simulink model "ProcessNetworkSimulation"  (R2015b)
settings: Solver=VariableStepAuto  StartTime=0.0  StopTime=1000.0  RelTol=1e-3
libraries: simulink x1, simeventslib x1
(part 1 of 21)
settings Model: Creator=tsprock3  LastModifiedBy=tsprock3

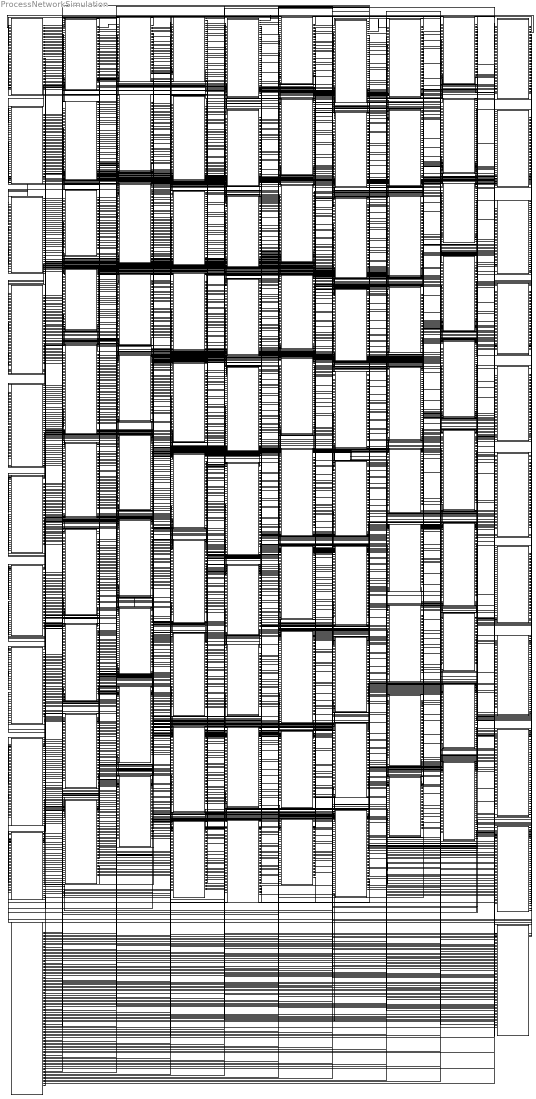
== system ProcessNetworkSimulation ==
  Arrival_Process : Subsystem
  Departure_Process : Subsystem
  Process_1 : Subsystem
  Process_10 : Subsystem
  Process_100 : Subsystem
  Process_11 : Subsystem
  Process_12 : Subsystem
  Process_13 : Subsystem
  Process_14 : Subsystem
  Process_15 : Subsystem
  Process_16 : Subsystem
  Process_17 : Subsystem
  Process_18 : Subsystem
  Process_19 : Subsystem
  Process_2 : Subsystem
  Process_20 : Subsystem
  Process_21 : Subsystem
  Process_22 : Subsystem
  Process_23 : Subsystem
  Process_24 : Subsystem
  Process_25 : Subsystem
  Process_26 : Subsystem
  Process_27 : Subsystem
  Process_28 : Subsystem
  Process_29 : Subsystem
  Process_3 : Subsystem
  Process_30 : Subsystem
  Process_31 : Subsystem
  Process_32 : Subsystem
  Process_33 : Subsystem
  Process_34 : Subsystem
  Process_35 : Subsystem
  Process_36 : Subsystem
  Process_37 : Subsystem
  Process_38 : Subsystem
  Process_39 : Subsystem
  Process_4 : Subsystem
  Process_40 : Subsystem
  Process_41 : Subsystem
  Process_42 : Subsystem
  Process_43 : Subsystem
  Process_44 : Subsystem
  Process_45 : Subsystem
  Process_46 : Subsystem
  Process_47 : Subsystem
  Process_48 : Subsystem
  Process_49 : Subsystem
  Process_5 : Subsystem
  Process_50 : Subsystem
  Process_51 : Subsystem
  Process_52 : Subsystem
  Process_53 : Subsystem
  Process_54 : Subsystem
  Process_55 : Subsystem
  Process_56 : Subsystem
  Process_57 : Subsystem
  Process_58 : Subsystem
  Process_59 : Subsystem
  Process_6 : Subsystem
  Process_60 : Subsystem
  Process_61 : Subsystem
  Process_62 : Subsystem
  Process_63 : Subsystem
  Process_64 : Subsystem
  Process_65 : Subsystem
  Process_66 : Subsystem
  Process_67 : Subsystem
  Process_68 : Subsystem
  Process_69 : Subsystem
  Process_7 : Subsystem
  Process_70 : Subsystem
  Process_71 : Subsystem
  Process_72 : Subsystem
  Process_73 : Subsystem
  Process_74 : Subsystem
  Process_75 : Subsystem
  Process_76 : Subsystem
  Process_77 : Subsystem
  Process_78 : Subsystem
  Process_79 : Subsystem
  Process_8 : Subsystem
  Process_80 : Subsystem
  Process_81 : Subsystem
  Process_82 : Subsystem
  Process_83 : Subsystem
  Process_84 : Subsystem
  Process_85 : Subsystem
  Process_86 : Subsystem
  Process_87 : Subsystem
  Process_88 : Subsystem
  Process_89 : Subsystem
  Process_9 : Subsystem
  Process_90 : Subsystem
  Process_91 : Subsystem
  Process_92 : Subsystem
  Process_93 : Subsystem
  Process_94 : Subsystem
  Process_95 : Subsystem
  Process_96 : Subsystem
  Process_97 : Subsystem
  Process_98 : Subsystem
  Process_99 : Subsystem
  connections:
  Process_1/RConn1 -- Process_1/LConn1
  Process_1/RConn2 -- Process_2/LConn1
  Process_1/RConn3 -- Process_4/LConn1
  Process_1/RConn4 -- Process_8/LConn1
  Process_1/RConn5 -- Process_10/LConn1
  Process_1/RConn6 -- Process_11/LConn1
  Process_1/RConn7 -- Process_16/LConn1
  Process_1/RConn8 -- Process_18/LConn1
  Process_1/RConn9 -- Process_23/LConn1
  Process_1/RConn10 -- Process_24/LConn1
  Process_1/RConn11 -- Process_25/LConn1
  Process_1/RConn12 -- Process_30/LConn1
  Process_1/RConn13 -- Process_33/LConn1
  Process_1/RConn14 -- Process_35/LConn1
  Process_1/RConn15 -- Process_38/LConn1
  Process_1/RConn16 -- Process_40/LConn1
  Process_1/RConn17 -- Process_45/LConn1
  Process_1/RConn18 -- Process_48/LConn1
  Process_1/RConn19 -- Process_54/LConn1
  Process_1/RConn20 -- Process_57/LConn1
  Process_1/RConn21 -- Process_58/LConn1
  Process_1/RConn22 -- Process_59/LConn1
  Process_1/RConn23 -- Process_64/LConn1
  Process_1/RConn24 -- Process_65/LConn1
  Process_1/RConn25 -- Process_67/LConn1
  Process_1/RConn26 -- Process_69/LConn1
  Process_1/RConn27 -- Process_71/LConn1
  Process_1/RConn28 -- Process_72/LConn1
  Process_1/RConn29 -- Process_74/LConn1
  Process_1/RConn30 -- Process_77/LConn1
  Process_1/RConn31 -- Process_81/LConn1
  Process_1/RConn32 -- Process_83/LConn1
  Process_1/RConn33 -- Process_93/LConn1
  Process_1/RConn34 -- Process_97/LConn1
  Process_1/RConn35 -- Process_99/LConn1
  Process_1/RConn36 -- Process_100/LConn1
  Process_2/RConn1 -- Process_1/LConn2
  Process_2/RConn2 -- Process_6/LConn1
  Process_2/RConn3 -- Process_15/LConn1
  Process_2/RConn4 -- Process_18/LConn2
  Process_2/RConn5 -- Process_19/LConn1
  Process_2/RConn6 -- Process_20/LConn1
  Process_2/RConn7 -- Process_22/LConn1
  Process_2/RConn8 -- Process_27/LConn1
  Process_2/RConn9 -- Process_30/LConn2
  Process_2/RConn10 -- Process_32/LConn1
  Process_2/RConn11 -- Process_33/LConn2
  Process_2/RConn12 -- Process_42/LConn1
  Process_2/RConn13 -- Process_45/LConn2
  Process_2/RConn14 -- Process_46/LConn1
  Process_2/RConn15 -- Process_52/LConn1
  Process_2/RConn16 -- Process_54/LConn2
  Process_2/RConn17 -- Process_56/LConn1
  Process_2/RConn18 -- Process_58/LConn2
  Process_2/RConn19 -- Process_59/LConn2
  Process_2/RConn20 -- Process_60/LConn1
  Process_2/RConn21 -- Process_67/LConn2
  Process_2/RConn22 -- Process_69/LConn2
  Process_2/RConn23 -- Process_82/LConn1
  Process_2/RConn24 -- Process_85/LConn1
  Process_2/RConn25 -- Process_91/LConn1
  Process_2/RConn26 -- Process_92/LConn1
  Process_2/RConn27 -- Process_93/LConn2
  Process_2/RConn28 -- Process_95/LConn1
  Process_2/RConn29 -- Process_96/LConn1
  Process_2/RConn30 -- Process_98/LConn1
  Process_2/RConn31 -- Process_99/LConn2
  Process_3/RConn1 -- Process_6/LConn2
  Process_3/RConn2 -- Process_11/LConn2
  Process_3/RConn3 -- Process_16/LConn2
  Process_3/RConn4 -- Process_28/LConn1
  Process_3/RConn5 -- Process_34/LConn1
  Process_3/RConn6 -- Process_35/LConn2
  Process_3/RConn7 -- Process_43/LConn1
  Process_3/RConn8 -- Process_44/LConn1
  Process_3/RConn9 -- Process_45/LConn3
  Process_3/RConn10 -- Process_51/LConn1
  Process_3/RConn11 -- Process_52/LConn2
  Process_3/RConn12 -- Process_55/LConn1
  Process_3/RConn13 -- Process_60/LConn2
  Process_3/RConn14 -- Process_62/LConn1
  Process_3/RConn15 -- Process_66/LConn1
  Process_3/RConn16 -- Process_68/LConn1
  Process_3/RConn17 -- Process_71/LConn2
  Process_3/RConn18 -- Process_75/LConn1
  Process_3/RConn19 -- Process_77/LConn2
  Process_3/RConn20 -- Process_79/LConn1
  Process_3/RConn21 -- Process_80/LConn1
  Process_3/RConn22 -- Process_83/LConn2
  Process_3/RConn23 -- Process_85/LConn2
  Process_3/RConn24 -- Process_88/LConn1
  Process_3/RConn25 -- Process_92/LConn2
  Process_3/RConn26 -- Process_95/LConn2
  Process_3/RConn27 -- Process_97/LConn2
  Process_3/RConn28 -- Process_98/LConn2
  Process_3/RConn29 -- Process_99/LConn3
  Process_3/RConn30 -- Process_100/LConn2
  Process_4/RConn1 -- Process_5/LConn1
  Process_4/RConn2 -- Process_6/LConn3
  Process_4/RConn3 -- Process_9/LConn1
  Process_4/RConn4 -- Process_11/LConn3
  Process_4/RConn5 -- Process_20/LConn2
  Process_4/RConn6 -- Process_22/LConn2
  Process_4/RConn7 -- Process_23/LConn2
  Process_4/RConn8 -- Process_29/LConn1
  Process_4/RConn9 -- Process_30/LConn3
  Process_4/RConn10 -- Process_33/LConn3
  Process_4/RConn11 -- Process_37/LConn1
  Process_4/RConn12 -- Process_39/LConn1
  Process_4/RConn13 -- Process_41/LConn1
  Process_4/RConn14 -- Process_42/LConn2
  Process_4/RConn15 -- Process_43/LConn2
  Process_4/RConn16 -- Process_44/LConn2
  Process_4/RConn17 -- Process_47/LConn1
  Process_4/RConn18 -- Process_49/LConn1
  Process_4/RConn19 -- Process_50/LConn1
  Process_4/RConn20 -- Process_53/LConn1
  Process_4/RConn21 -- Process_57/LConn2
  Process_4/RConn22 -- Process_64/LConn2
  Process_4/RConn23 -- Process_70/LConn1
  Process_4/RConn24 -- Process_72/LConn2
  Process_4/RConn25 -- Process_74/LConn2
  Process_4/RConn26 -- Process_77/LConn3
  Process_4/RConn27 -- Process_81/LConn2
  Process_4/RConn28 -- Process_83/LConn3
  Process_4/RConn29 -- Process_84/LConn1
  Process_4/RConn30 -- Process_86/LConn1
  Process_4/RConn31 -- Process_89/LConn1
  Process_4/RConn32 -- Process_90/LConn1
  Process_4/RConn33 -- Process_91/LConn2
  Process_4/RConn34 -- Process_94/LConn1
  Process_4/RConn35 -- Process_95/LConn3
  Process_4/RConn36 -- Process_100/LConn3
  Process_5/RConn1 -- Process_5/LConn2
  Process_5/RConn2 -- Process_8/LConn2
  Process_5/RConn3 -- Process_9/LConn2
  Process_5/RConn4 -- Process_13/LConn1
  Process_5/RConn5 -- Process_15/LConn2
  Process_5/RConn6 -- Process_16/LConn3
  Process_5/RConn7 -- Process_17/LConn1
  Process_5/RConn8 -- Process_21/LConn1
  Process_5/RConn9 -- Process_30/LConn4
  Process_5/RConn10 -- Process_32/LConn2
  Process_5/RConn11 -- Process_35/LConn3
  Process_5/RConn12 -- Process_37/LConn2
  Process_5/RConn13 -- Process_38/LConn2
  Process_5/RConn14 -- Process_45/LConn4
  Process_5/RConn15 -- Process_48/LConn2
  Process_5/RConn16 -- Process_53/LConn2
  Process_5/RConn17 -- Process_56/LConn2
  Process_5/RConn18 -- Process_58/LConn3
  Process_5/RConn19 -- Process_59/LConn3
  Process_5/RConn20 -- Process_62/LConn2
  Process_5/RConn21 -- Process_63/LConn1
  Process_5/RConn22 -- Process_64/LConn3
  Process_5/RConn23 -- Process_68/LConn2
  Process_5/RConn24 -- Process_72/LConn3
  Process_5/RConn25 -- Process_75/LConn2
  Process_5/RConn26 -- Process_76/LConn1
  Process_5/RConn27 -- Process_79/LConn2
  Process_5/RConn28 -- Process_81/LConn3
  Process_5/RConn29 -- Process_82/LConn2
  Process_5/RConn30 -- Process_83/LConn4
  Process_5/RConn31 -- Process_88/LConn2
  Process_5/RConn32 -- Process_90/LConn2
  Process_5/RConn33 -- Process_94/LConn2
  Process_5/RConn34 -- Process_95/LConn4
  Process_5/RConn35 -- Process_96/LConn2
  Process_6/RConn1 -- Process_1/LConn3
  Process_6/RConn2 -- Process_2/LConn2
  Process_6/RConn3 -- Process_4/LConn2
  Process_6/RConn4 -- Process_5/LConn3
  Process_6/RConn5 -- Process_6/LConn4
  Process_6/RConn6 -- Process_7/LConn1
  Process_6/RConn7 -- Process_8/LConn3
  Process_6/RConn8 -- Process_11/LConn4
  Process_6/RConn9 -- Process_14/LConn1
  Process_6/RConn10 -- Process_16/LConn4
  Process_6/RConn11 -- Process_17/LConn2
  Process_6/RConn12 -- Process_18/LConn3
  Process_6/RConn13 -- Process_19/LConn2
  Process_6/RConn14 -- Process_21/LConn2
  Process_6/RConn15 -- Process_29/LConn2
  Process_6/RConn16 -- Process_36/LConn1
  Process_6/RConn17 -- Process_38/LConn3
  Process_6/RConn18 -- Process_43/LConn3
  Process_6/RConn19 -- Process_44/LConn3
  Process_6/RConn20 -- Process_46/LConn2
  Process_6/RConn21 -- Process_47/LConn2
  Process_6/RConn22 -- Process_50/LConn2
  Process_6/RConn23 -- Process_58/LConn4
  Process_6/RConn24 -- Process_59/LConn4
  Process_6/RConn25 -- Process_60/LConn3
  Process_6/RConn26 -- Process_61/LConn1
  Process_6/RConn27 -- Process_63/LConn2
  Process_6/RConn28 -- Process_66/LConn2
  Process_6/RConn29 -- Process_67/LConn3
  Process_6/RConn30 -- Process_68/LConn3
  Process_6/RConn31 -- Process_77/LConn4
  Process_6/RConn32 -- Process_83/LConn5
  Process_6/RConn33 -- Process_85/LConn3
  Process_6/RConn34 -- Process_86/LConn2
  Process_6/RConn35 -- Process_89/LConn2
  Process_6/RConn36 -- Process_90/LConn3
  Process_6/RConn37 -- Process_97/LConn3
  Process_6/RConn38 -- Process_98/LConn3
  Process_7/RConn1 -- Process_2/LConn3
  Process_7/RConn2 -- Process_3/LConn1
  Process_7/RConn3 -- Process_7/LConn2
  Process_7/RConn4 -- Process_9/LConn3
  Process_7/RConn5 -- Process_16/LConn5
  Process_7/RConn6 -- Process_18/LConn4
  Process_7/RConn7 -- Process_20/LConn3
  Process_7/RConn8 -- Process_21/LConn3
  Process_7/RConn9 -- Process_27/LConn2
  Process_7/RConn10 -- Process_29/LConn3
  Process_7/RConn11 -- Process_32/LConn3
  Process_7/RConn12 -- Process_33/LConn4
  Process_7/RConn13 -- Process_35/LConn4
  Process_7/RConn14 -- Process_38/LConn4
  Process_7/RConn15 -- Process_39/LConn2
  Process_7/RConn16 -- Process_40/LConn2
  Process_7/RConn17 -- Process_41/LConn2
  Process_7/RConn18 -- Process_42/LConn3
  Process_7/RConn19 -- Process_46/LConn3
  Process_7/RConn20 -- Process_47/LConn3
  Process_7/RConn21 -- Process_50/LConn3
  Process_7/RConn22 -- Process_51/LConn2
  Process_7/RConn23 -- Process_52/LConn3
  Process_7/RConn24 -- Process_56/LConn3
  Process_7/RConn25 -- Process_59/LConn5
  Process_7/RConn26 -- Process_60/LConn4
  Process_7/RConn27 -- Process_61/LConn2
  Process_7/RConn28 -- Process_62/LConn3
  Process_7/RConn29 -- Process_64/LConn4
  Process_7/RConn30 -- Process_66/LConn3
  Process_7/RConn31 -- Process_67/LConn4
  Process_7/RConn32 -- Process_74/LConn3
  Process_7/RConn33 -- Process_75/LConn3
  Process_7/RConn34 -- Process_77/LConn5
  Process_7/RConn35 -- Process_79/LConn3
  Process_7/RConn36 -- Process_80/LConn2
  Process_7/RConn37 -- Process_82/LConn3
  Process_7/RConn38 -- Process_83/LConn6
  Process_7/RConn39 -- Process_89/LConn3
  Process_7/RConn40 -- Process_90/LConn4
  Process_7/RConn41 -- Process_93/LConn3
  Process_8/RConn1 -- Process_3/LConn2
  Process_8/RConn2 -- Process_6/LConn5
  Process_8/RConn3 -- Process_12/LConn1
  Process_8/RConn4 -- Process_13/LConn2
  Process_8/RConn5 -- Process_16/LConn6
  Process_8/RConn6 -- Process_23/LConn3
  Process_8/RConn7 -- Process_27/LConn3
  Process_8/RConn8 -- Process_30/LConn5
  Process_8/RConn9 -- Process_36/LConn2
  Process_8/RConn10 -- Process_37/LConn3
  Process_8/RConn11 -- Process_38/LConn5
  Process_8/RConn12 -- Process_41/LConn3
  Process_8/RConn13 -- Process_42/LConn4
  Process_8/RConn14 -- Process_43/LConn4
  Process_8/RConn15 -- Process_46/LConn4
  Process_8/RConn16 -- Process_50/LConn4
  Process_8/RConn17 -- Process_53/LConn3
  Process_8/RConn18 -- Process_54/LConn3
  Process_8/RConn19 -- Process_56/LConn4
  Process_8/RConn20 -- Process_60/LConn5
  Process_8/RConn21 -- Process_68/LConn4
  Process_8/RConn22 -- Process_71/LConn3
  Process_8/RConn23 -- Process_73/LConn1
  Process_8/RConn24 -- Process_74/LConn4
  Process_8/RConn25 -- Process_76/LConn2
  Process_8/RConn26 -- Process_77/LConn6
  Process_8/RConn27 -- Process_79/LConn4
  Process_8/RConn28 -- Process_80/LConn3
  Process_8/RConn29 -- Process_86/LConn3
  Process_8/RConn30 -- Process_90/LConn5
  Process_8/RConn31 -- Process_91/LConn3
  Process_8/RConn32 -- Process_95/LConn5
  Process_8/RConn33 -- Process_97/LConn4
  Process_9/RConn1 -- Process_2/LConn4
  Process_9/RConn2 -- Process_3/LConn3
  Process_9/RConn3 -- Process_4/LConn3
  Process_9/RConn4 -- Process_6/LConn6
  Process_9/RConn5 -- Process_10/LConn2
  Process_9/RConn6 -- Process_11/LConn5
  Process_9/RConn7 -- Process_13/LConn3
  Process_9/RConn8 -- Process_14/LConn2
  Process_9/RConn9 -- Process_15/LConn3
  Process_9/RConn10 -- Process_23/LConn4
  Process_9/RConn11 -- Process_24/LConn2
  Process_9/RConn12 -- Process_26/LConn1
  Process_9/RConn13 -- Process_27/LConn4
  Process_9/RConn14 -- Process_28/LConn2
  Process_9/RConn15 -- Process_30/LConn6
  Process_9/RConn16 -- Process_31/LConn1
  Process_9/RConn17 -- Process_32/LConn4
  Process_9/RConn18 -- Process_34/LConn2
  Process_9/RConn19 -- Process_36/LConn3
  Process_9/RConn20 -- Process_37/LConn4
  Process_9/RConn21 -- Process_38/LConn6
  Process_9/RConn22 -- Process_40/LConn3
  Process_9/RConn23 -- Process_41/LConn4
  Process_9/RConn24 -- Process_42/LConn5
  Process_9/RConn25 -- Process_44/LConn4
  Process_9/RConn26 -- Process_49/LConn2
  Process_9/RConn27 -- Process_55/LConn2
  Process_9/RConn28 -- Process_56/LConn5
  Process_9/RConn29 -- Process_58/LConn5
  Process_9/RConn30 -- Process_61/LConn3
  Process_9/RConn31 -- Process_62/LConn4
  Process_9/RConn32 -- Process_65/LConn2
  Process_9/RConn33 -- Process_71/LConn4
  Process_9/RConn34 -- Process_76/LConn3
  Process_9/RConn35 -- Process_80/LConn4
  Process_9/RConn36 -- Process_82/LConn4
  Process_9/RConn37 -- Process_83/LConn7
  Process_9/RConn38 -- Process_88/LConn3
  Process_9/RConn39 -- Process_92/LConn3
  Process_9/RConn40 -- Process_93/LConn4
  Process_9/RConn41 -- Process_98/LConn4
  Process_9/RConn42 -- Process_99/LConn4
  Process_10/RConn1 -- Process_2/LConn5
  Process_10/RConn2 -- Process_4/LConn4
  Process_10/RConn3 -- Process_5/LConn4
  Process_10/RConn4 -- Process_8/LConn4
  Process_10/RConn5 -- Process_9/LConn4
  Process_10/RConn6 -- Process_11/LConn6
  Process_10/RConn7 -- Process_14/LConn3
  Process_10/RConn8 -- Process_18/LConn5
  Process_10/RConn9 -- Process_22/LConn3
  Process_10/RConn10 -- Process_24/LConn3
  Process_10/RConn11 -- Process_25/LConn2
  Process_10/RConn12 -- Process_26/LConn2
  Process_10/RConn13 -- Process_29/LConn4
  Process_10/RConn14 -- Process_33/LConn5
  Process_10/RConn15 -- Process_37/LConn5
  Process_10/RConn16 -- Process_38/LConn7
  Process_10/RConn17 -- Process_41/LConn5
  Process_10/RConn18 -- Process_42/LConn6
  Process_10/RConn19 -- Process_43/LConn5
  Process_10/RConn20 -- Process_48/LConn3
  Process_10/RConn21 -- Process_49/LConn3
  Process_10/RConn22 -- Process_50/LConn5
  Process_10/RConn23 -- Process_59/LConn6
  Process_10/RConn24 -- Process_63/LConn3
  Process_10/RConn25 -- Process_68/LConn5
  Process_10/RConn26 -- Process_70/LConn2
  Process_10/RConn27 -- Process_72/LConn4
  Process_10/RConn28 -- Process_75/LConn4
  Process_10/RConn29 -- Process_76/LConn4
  Process_10/RConn30 -- Process_79/LConn5
  Process_10/RConn31 -- Process_80/LConn5
  Process_10/RConn32 -- Process_81/LConn4
  Process_10/RConn33 -- Process_83/LConn8
  Process_10/RConn34 -- Process_84/LConn2
  Process_10/RConn35 -- Process_89/LConn4
  Process_10/RConn36 -- Process_90/LConn6
  Process_10/RConn37 -- Process_91/LConn4
  Process_10/RConn38 -- Process_92/LConn4
  Process_10/RConn39 -- Process_93/LConn5
  Process_10/RConn40 -- Process_95/LConn6
  Process_11/RConn1 -- Process_6/LConn7
  Process_11/RConn2 -- Process_7/LConn3
  Process_11/RConn3 -- Process_9/LConn5
  Process_11/RConn4 -- Process_13/LConn4
  Process_11/RConn5 -- Process_15/LConn4
  Process_11/RConn6 -- Process_18/LConn6
  Process_11/RConn7 -- Process_21/LConn4
  Process_11/RConn8 -- Process_28/LConn3
  Process_11/RConn9 -- Process_29/LConn5
  Process_11/RConn10 -- Process_33/LConn6
  Process_11/RConn11 -- Process_36/LConn4
  Process_11/RConn12 -- Process_40/LConn4
  Process_11/RConn13 -- Process_41/LConn6
  Process_11/RConn14 -- Process_42/LConn7
  Process_11/RConn15 -- Process_44/LConn5
  Process_11/RConn16 -- Process_45/LConn5
  Process_11/RConn17 -- Process_46/LConn5
  Process_11/RConn18 -- Process_47/LConn4
  Process_11/RConn19 -- Process_49/LConn4
  Process_11/RConn20 -- Process_53/LConn4
  Process_11/RConn21 -- Process_55/LConn3
  Process_11/RConn22 -- Process_59/LConn7
  Process_11/RConn23 -- Process_61/LConn4
  Process_11/RConn24 -- Process_67/LConn5
  Process_11/RConn25 -- Process_68/LConn6
  Process_11/RConn26 -- Process_70/LConn3
  Process_11/RConn27 -- Process_72/LConn5
  Process_11/RConn28 -- Process_73/LConn2
  Process_11/RConn29 -- Process_74/LConn5
  Process_11/RConn30 -- Process_77/LConn7
  Process_11/RConn31 -- Process_82/LConn5
  Process_11/RConn32 -- Process_83/LConn9
  Process_11/RConn33 -- Process_93/LConn6
  Process_11/RConn34 -- Process_96/LConn3
  Process_11/RConn35 -- Process_99/LConn5
  Process_11/RConn36 -- Process_100/LConn4
  Process_12/RConn1 -- Process_1/LConn4
  Process_12/RConn2 -- Process_4/LConn5
  Process_12/RConn3 -- Process_6/LConn8
  Process_12/RConn4 -- Process_7/LConn4
  Process_12/RConn5 -- Process_9/LConn6
  Process_12/RConn6 -- Process_10/LConn3
  Process_12/RConn7 -- Process_13/LConn5
  Process_12/RConn8 -- Process_14/LConn4
  Process_12/RConn9 -- Process_16/LConn7
  Process_12/RConn10 -- Process_19/LConn3
  Process_12/RConn11 -- Process_23/LConn5
  Process_12/RConn12 -- Process_28/LConn4
  Process_12/RConn13 -- Process_30/LConn7
  Process_12/RConn14 -- Process_35/LConn5
  Process_12/RConn15 -- Process_36/LConn5
  Process_12/RConn16 -- Process_41/LConn7
  Process_12/RConn17 -- Process_44/LConn6
  Process_12/RConn18 -- Process_46/LConn6
  Process_12/RConn19 -- Process_47/LConn5
  Process_12/RConn20 -- Process_50/LConn6
  Process_12/RConn21 -- Process_52/LConn4
  Process_12/RConn22 -- Process_55/LConn4
  Process_12/RConn23 -- Process_56/LConn6
  Process_12/RConn24 -- Process_57/LConn3
  Process_12/RConn25 -- Process_58/LConn6
  Process_12/RConn26 -- Process_61/LConn5
  Process_12/RConn27 -- Process_62/LConn5
  Process_12/RConn28 -- Process_65/LConn3
  Process_12/RConn29 -- Process_71/LConn5
  Process_12/RConn30 -- Process_72/LConn6
  Process_12/RConn31 -- Process_73/LConn3
  Process_12/RConn32 -- Process_74/LConn6
  Process_12/RConn33 -- Process_78/LConn1
  Process_12/RConn34 -- Process_80/LConn6
  Process_12/RConn35 -- Process_83/LConn10
  Process_12/RConn36 -- Process_89/LConn5
  Process_12/RConn37 -- Process_91/LConn5
  Process_12/RConn38 -- Process_92/LConn5
  Process_12/RConn39 -- Process_93/LConn7
  Process_12/RConn40 -- Process_99/LConn6
  Process_13/RConn1 -- Process_6/LConn9
  Process_13/RConn2 -- Process_7/LConn5
  Process_13/RConn3 -- Process_11/LConn7
  Process_13/RConn4 -- Process_17/LConn3
  Process_13/RConn5 -- Process_18/LConn7
  Process_13/RConn6 -- Process_19/LConn4
  Process_13/RConn7 -- Process_20/LConn4
  Process_13/RConn8 -- Process_22/LConn4
  Process_13/RConn9 -- Process_24/LConn4
  Process_13/RConn10 -- Process_25/LConn3
  Process_13/RConn11 -- Process_26/LConn3
  Process_13/RConn12 -- Process_28/LConn5
  Process_13/RConn13 -- Process_30/LConn8
  Process_13/RConn14 -- Process_31/LConn2
  Process_13/RConn15 -- Process_33/LConn7
  Process_13/RConn16 -- Process_35/LConn6
  Process_13/RConn17 -- Process_36/LConn6
  Process_13/RConn18 -- Process_38/LConn8
  Process_13/RConn19 -- Process_39/LConn3
  Process_13/RConn20 -- Process_40/LConn5
  Process_13/RConn21 -- Process_45/LConn6
  Process_13/RConn22 -- Process_48/LConn4
  Process_13/RConn23 -- Process_50/LConn7
  Process_13/RConn24 -- Process_55/LConn5
  Process_13/RConn25 -- Process_62/LConn6
  Process_13/RConn26 -- Process_65/LConn4
  Process_13/RConn27 -- Process_66/LConn4
  Process_13/RConn28 -- Process_68/LConn7
  Process_13/RConn29 -- Process_69/LConn3
  Process_13/RConn30 -- Process_70/LConn4
  Process_13/RConn31 -- Process_71/LConn6
  Process_13/RConn32 -- Process_72/LConn7
  Process_13/RConn33 -- Process_75/LConn5
  Process_13/RConn34 -- Process_76/LConn5
  Process_13/RConn35 -- Process_80/LConn7
  Process_13/RConn36 -- Process_82/LConn6
  Process_13/RConn37 -- Process_88/LConn4
  Process_13/RConn38 -- Process_89/LConn6
  Process_13/RConn39 -- Process_97/LConn5
  Process_13/RConn40 -- Process_98/LConn5
  Process_13/RConn41 -- Process_99/LConn7
  Process_14/RConn1 -- Process_3/LConn4
  Process_14/RConn2 -- Process_6/LConn10
  Process_14/RConn3 -- Process_7/LConn6
  Process_14/RConn4 -- Process_8/LConn5
  Process_14/RConn5 -- Process_9/LConn7
  Process_14/RConn6 -- Process_12/LConn2
  Process_14/RConn7 -- Process_13/LConn6
  Process_14/RConn8 -- Process_16/LConn8
  Process_14/RConn9 -- Process_18/LConn8
  Process_14/RConn10 -- Process_21/LConn5
  Process_14/RConn11 -- Process_23/LConn6
  Process_14/RConn12 -- Process_25/LConn4
  Process_14/RConn13 -- Process_26/LConn4
  Process_14/RConn14 -- Process_27/LConn5
  Process_14/RConn15 -- Process_29/LConn6
  Process_14/RConn16 -- Process_31/LConn3
  Process_14/RConn17 -- Process_40/LConn6
  Process_14/RConn18 -- Process_41/LConn8
  Process_14/RConn19 -- Process_43/LConn6
  Process_14/RConn20 -- Process_50/LConn8
  Process_14/RConn21 -- Process_51/LConn3
  Process_14/RConn22 -- Process_53/LConn5
  Process_14/RConn23 -- Process_56/LConn7
  Process_14/RConn24 -- Process_57/LConn4
  Process_14/RConn25 -- Process_58/LConn7
  Process_14/RConn26 -- Process_60/LConn6
  Process_14/RConn27 -- Process_61/LConn6
  Process_14/RConn28 -- Process_65/LConn5
  Process_14/RConn29 -- Process_66/LConn5
  Process_14/RConn30 -- Process_71/LConn7
  Process_14/RConn31 -- Process_74/LConn7
  Process_14/RConn32 -- Process_82/LConn7
  Process_14/RConn33 -- Process_83/LConn11
  Process_14/RConn34 -- Process_84/LConn3
  Process_14/RConn35 -- Process_89/LConn7
  Process_14/RConn36 -- Process_90/LConn7
  Process_14/RConn37 -- Process_91/LConn6
  Process_14/RConn38 -- Process_98/LConn6
  Process_14/RConn39 -- Process_99/LConn8
  Process_15/RConn1 -- Process_3/LConn5
  Process_15/RConn2 -- Process_4/LConn6
  Process_15/RConn3 -- Process_5/LConn5
  Process_15/RConn4 -- Process_15/LConn5
  Process_15/RConn5 -- Process_16/LConn9
  Process_15/RConn6 -- Process_17/LConn4
  Process_15/RConn7 -- Process_19/LConn5
  Process_15/RConn8 -- Process_25/LConn5
  Process_15/RConn9 -- Process_27/LConn6
  Process_15/RConn10 -- Process_30/LConn9
  Process_15/RConn11 -- Process_37/LConn6
  Process_15/RConn12 -- Process_39/LConn4
  Process_15/RConn13 -- Process_40/LConn7
  Process_15/RConn14 -- Process_41/LConn9
  Process_15/RConn15 -- Process_43/LConn7
  Process_15/RConn16 -- Process_46/LConn7
  Process_15/RConn17 -- Process_48/LConn5
  Process_15/RConn18 -- Process_49/LConn5
  Process_15/RConn19 -- Process_50/LConn9
  Process_15/RConn20 -- Process_54/LConn4
  Process_15/RConn21 -- Process_55/LConn6
  Process_15/RConn22 -- Process_56/LConn8
  Process_15/RConn23 -- Process_59/LConn8
  Process_15/RConn24 -- Process_60/LConn7
  Process_15/RConn25 -- Process_61/LConn7
  Process_15/RConn26 -- Process_63/LConn4
  Process_15/RConn27 -- Process_65/LConn6
  Process_15/RConn28 -- Process_66/LConn6
  Process_15/RConn29 -- Process_69/LConn4
  Process_15/RConn30 -- Process_73/LConn4
  Process_15/RConn31 -- Process_75/LConn6
  Process_15/RConn32 -- Process_82/LConn8
  Process_15/RConn33 -- Process_86/LConn4
  Process_15/RConn34 -- Process_87/LConn1
  Process_15/RConn35 -- Process_94/LConn3
  Process_15/RConn36 -- Process_98/LConn7
  Process_15/RConn37 -- Process_99/LConn9
  Process_16/RConn1 -- Process_4/LConn7
  Process_16/RConn2 -- Process_8/LConn6
  Process_16/RConn3 -- Process_9/LConn8
  Process_16/RConn4 -- Process_10/LConn4
  Process_16/RConn5 -- Process_12/LConn3
  Process_16/RConn6 -- Process_13/LConn7
  Process_16/RConn7 -- Process_16/LConn10
  Process_16/RConn8 -- Process_17/LConn5
  Process_16/RConn9 -- Process_19/LConn6
  Process_16/RConn10 -- Process_22/LConn5
  Process_16/RConn11 -- Process_23/LConn7
  Process_16/RConn12 -- Process_25/LConn6
  Process_16/RConn13 -- Process_26/LConn5
  Process_16/RConn14 -- Process_30/LConn10
  Process_16/RConn15 -- Process_42/LConn8
  Process_16/RConn16 -- Process_48/LConn6
  Process_16/RConn17 -- Process_49/LConn6
  Process_16/RConn18 -- Process_50/LConn10
  Process_16/RConn19 -- Process_51/LConn4
  Process_16/RConn20 -- Process_52/LConn5
  Process_16/RConn21 -- Process_55/LConn7
  Process_16/RConn22 -- Process_57/LConn5
  Process_16/RConn23 -- Process_58/LConn8
  Process_16/RConn24 -- Process_60/LConn8
  Process_16/RConn25 -- Process_61/LConn8
  Process_16/RConn26 -- Process_66/LConn7
  Process_16/RConn27 -- Process_69/LConn5
  Process_16/RConn28 -- Process_71/LConn8
  Process_16/RConn29 -- Process_75/LConn7
  Process_16/RConn30 -- Process_79/LConn6
  Process_16/RConn31 -- Process_81/LConn5
  Process_16/RConn32 -- Process_82/LConn9
  Process_16/RConn33 -- Process_83/LConn12
  Process_16/RConn34 -- Process_86/LConn5
  Process_16/RConn35 -- Process_87/LConn2
  Process_16/RConn36 -- Process_94/LConn4
  Process_16/RConn37 -- Process_96/LConn4
  Process_16/RConn38 -- Process_98/LConn8
  Process_16/RConn39 -- Process_99/LConn10
  Process_17/RConn1 -- Process_1/LConn5
  Process_17/RConn2 -- Process_3/LConn6
  Process_17/RConn3 -- Process_7/LConn7
  Process_17/RConn4 -- Process_10/LConn5
  Process_17/RConn5 -- Process_14/LConn5
  Process_17/RConn6 -- Process_17/LConn6
  Process_17/RConn7 -- Process_22/LConn6
  Process_17/RConn8 -- Process_23/LConn8
  Process_17/RConn9 -- Process_26/LConn6
  Process_17/RConn10 -- Process_30/LConn11
  Process_17/RConn11 -- Process_33/LConn8
  Process_17/RConn12 -- Process_34/LConn3
  Process_17/RConn13 -- Process_38/LConn9
  Process_17/RConn14 -- Process_41/LConn10
  Process_17/RConn15 -- Process_53/LConn6
  Process_17/RConn16 -- Process_57/LConn6
  Process_17/RConn17 -- Process_58/LConn9
  Process_17/RConn18 -- Process_64/LConn5
  Process_17/RConn19 -- Process_70/LConn5
  Process_17/RConn20 -- Process_76/LConn6
  Process_17/RConn21 -- Process_79/LConn7
  Process_17/RConn22 -- Process_80/LConn8
  Process_17/RConn23 -- Process_82/LConn10
  Process_17/RConn24 -- Process_83/LConn13
  Process_17/RConn25 -- Process_89/LConn8
  Process_17/RConn26 -- Process_93/LConn8
  Process_17/RConn27 -- Process_94/LConn5
  Process_17/RConn28 -- Process_96/LConn5
  Process_17/RConn29 -- Process_97/LConn6
  Process_17/RConn30 -- Process_98/LConn9
  Process_17/RConn31 -- Process_99/LConn11
  Process_17/RConn32 -- Process_100/LConn5
  Process_18/RConn1 -- Process_2/LConn6
  Process_18/RConn2 -- Process_10/LConn6
  Process_18/RConn3 -- Process_15/LConn6
  Process_18/RConn4 -- Process_17/LConn7
  Process_18/RConn5 -- Process_21/LConn6
  Process_18/RConn6 -- Process_22/LConn7
  Process_18/RConn7 -- Process_26/LConn7
  Process_18/RConn8 -- Process_27/LConn7
  Process_18/RConn9 -- Process_28/LConn6
  Process_18/RConn10 -- Process_31/LConn4
  Process_18/RConn11 -- Process_32/LConn5
  Process_18/RConn12 -- Process_34/LConn4
  Process_18/RConn13 -- Process_36/LConn7
  Process_18/RConn14 -- Process_44/LConn7
  Process_18/RConn15 -- Process_45/LConn7
  Process_18/RConn16 -- Process_47/LConn6
  Process_18/RConn17 -- Process_51/LConn5
  Process_18/RConn18 -- Process_52/LConn6
  Process_18/RConn19 -- Process_53/LConn7
  Process_18/RConn20 -- Process_61/LConn9
  Process_18/RConn21 -- Process_68/LConn8
  Process_18/RConn22 -- Process_69/LConn6
  Process_18/RConn23 -- Process_70/LConn6
  Process_18/RConn24 -- Process_71/LConn9
  Process_18/RConn25 -- Process_74/LConn8
  Process_18/RConn26 -- Process_76/LConn7
  Process_18/RConn27 -- Process_78/LConn2
  Process_18/RConn28 -- Process_81/LConn6
  Process_18/RConn29 -- Process_83/LConn14
  Process_18/RConn30 -- Process_86/LConn6
  Process_18/RConn31 -- Process_87/LConn3
  Process_18/RConn32 -- Process_90/LConn8
  Process_18/RConn33 -- Process_92/LConn6
  Process_18/RConn34 -- Process_94/LConn6
  Process_18/RConn35 -- Process_96/LConn6
  Process_18/RConn36 -- Process_98/LConn10
  Process_19/RConn1 -- Process_1/LConn6
  Process_19/RConn2 -- Process_5/LConn6
  Process_19/RConn3 -- Process_9/LConn9
  Process_19/RConn4 -- Process_11/LConn8
  Process_19/RConn5 -- Process_15/LConn7
  Process_19/RConn6 -- Process_17/LConn8
  Process_19/RConn7 -- Process_18/LConn9
  Process_19/RConn8 -- Process_23/LConn9
  Process_19/RConn9 -- Process_29/LConn7
  Process_19/RConn10 -- Process_30/LConn12
  Process_19/RConn11 -- Process_34/LConn5
  Process_19/RConn12 -- Process_36/LConn8
  Process_19/RConn13 -- Process_41/LConn11
  Process_19/RConn14 -- Process_43/LConn8
  Process_19/RConn15 -- Process_44/LConn8
  Process_19/RConn16 -- Process_50/LConn11
  Process_19/RConn17 -- Process_51/LConn6
  Process_19/RConn18 -- Process_52/LConn7
  Process_19/RConn19 -- Process_56/LConn9
  Process_19/RConn20 -- Process_58/LConn10
  Process_19/RConn21 -- Process_59/LConn9
  Process_19/RConn22 -- Process_61/LConn10
  Process_19/RConn23 -- Process_63/LConn5
  Process_19/RConn24 -- Process_65/LConn7
  Process_19/RConn25 -- Process_69/LConn7
  Process_19/RConn26 -- Process_74/LConn9
  Process_19/RConn27 -- Process_75/LConn8
  Process_19/RConn28 -- Process_77/LConn8
  Process_19/RConn29 -- Process_79/LConn8
  Process_19/RConn30 -- Process_81/LConn7
  Process_19/RConn31 -- Process_83/LConn15
  Process_19/RConn32 -- Process_84/LConn4
  Process_19/RConn33 -- Process_85/LConn4
  Process_19/RConn34 -- Process_86/LConn7
  Process_19/RConn35 -- Process_88/LConn5
  Process_19/RConn36 -- Process_90/LConn9
  Process_19/RConn37 -- Process_91/LConn7
  Process_19/RConn38 -- Process_97/LConn7
  Process_19/RConn39 -- Process_98/LConn11
  Process_19/RConn40 -- Process_99/LConn12
  Process_19/RConn41 -- Process_100/LConn6
  Process_20/RConn1 -- Process_1/LConn7
  Process_20/RConn2 -- Process_2/LConn7
  Process_20/RConn3 -- Process_4/LConn8
  Process_20/RConn4 -- Process_6/LConn11
  Process_20/RConn5 -- Process_8/LConn7
  Process_20/RConn6 -- Process_9/LConn10
  Process_20/RConn7 -- Process_12/LConn4
  Process_20/RConn8 -- Process_16/LConn11
  Process_20/RConn9 -- Process_17/LConn9
  Process_20/RConn10 -- Process_29/LConn8
  Process_20/RConn11 -- Process_32/LConn6
  Process_20/RConn12 -- Process_34/LConn6
  Process_20/RConn13 -- Process_37/LConn7
  Process_20/RConn14 -- Process_40/LConn8
  Process_20/RConn15 -- Process_42/LConn9
  Process_20/RConn16 -- Process_43/LConn9
  Process_20/RConn17 -- Process_46/LConn8
  Process_20/RConn18 -- Process_51/LConn7
  Process_20/RConn19 -- Process_53/LConn8
  Process_20/RConn20 -- Process_54/LConn5
  Process_20/RConn21 -- Process_55/LConn8
  Process_20/RConn22 -- Process_57/LConn7
  Process_20/RConn23 -- Process_59/LConn10
  Process_20/RConn24 -- Process_62/LConn7
  Process_20/RConn25 -- Process_68/LConn9
  Process_20/RConn26 -- Process_69/LConn8
  Process_20/RConn27 -- Process_71/LConn10
  Process_20/RConn28 -- Process_78/LConn3
  Process_20/RConn29 -- Process_79/LConn9
  Process_20/RConn30 -- Process_82/LConn11
  Process_20/RConn31 -- Process_85/LConn5
  Process_20/RConn32 -- Process_87/LConn4
  Process_20/RConn33 -- Process_88/LConn6
  Process_20/RConn34 -- Process_91/LConn8
  Process_20/RConn35 -- Process_92/LConn7
  Process_20/RConn36 -- Process_93/LConn9
  Process_20/RConn37 -- Process_94/LConn7
  Process_20/RConn38 -- Process_96/LConn7
  Process_20/RConn39 -- Process_98/LConn12
  Process_20/RConn40 -- Process_99/LConn13
  Process_20/RConn41 -- Process_100/LConn7
  Process_21/RConn1 -- Process_7/LConn8
  Process_21/RConn2 -- Process_10/LConn7
  Process_21/RConn3 -- Process_12/LConn5
  Process_21/RConn4 -- Process_15/LConn8
  Process_21/RConn5 -- Process_21/LConn7
  Process_21/RConn6 -- Process_22/LConn8
  Process_21/RConn7 -- Process_23/LConn10
  Process_21/RConn8 -- Process_24/LConn5
  Process_21/RConn9 -- Process_26/LConn8
  Process_21/RConn10 -- Process_28/LConn7
  Process_21/RConn11 -- Process_31/LConn5
  Process_21/RConn12 -- Process_34/LConn7
  Process_21/RConn13 -- Process_37/LConn8
  Process_21/RConn14 -- Process_39/LConn5
  Process_21/RConn15 -- Process_40/LConn9
  Process_21/RConn16 -- Process_43/LConn10
  Process_21/RConn17 -- Process_46/LConn9
  Process_21/RConn18 -- Process_47/LConn7
  Process_21/RConn19 -- Process_48/LConn7
  Process_21/RConn20 -- Process_53/LConn9
  Process_21/RConn21 -- Process_59/LConn11
  Process_21/RConn22 -- Process_62/LConn8
  Process_21/RConn23 -- Process_64/LConn6
  Process_21/RConn24 -- Process_66/LConn8
  Process_21/RConn25 -- Process_70/LConn7
  Process_21/RConn26 -- Process_73/LConn5
  Process_21/RConn27 -- Process_79/LConn10
  Process_21/RConn28 -- Process_81/LConn8
  Process_21/RConn29 -- Process_87/LConn5
  Process_21/RConn30 -- Process_88/LConn7
  Process_21/RConn31 -- Process_91/LConn9
  Process_21/RConn32 -- Process_93/LConn10
  Process_21/RConn33 -- Process_99/LConn14
  Process_22/RConn1 -- Process_3/LConn7
  Process_22/RConn2 -- Process_6/LConn12
  Process_22/RConn3 -- Process_8/LConn8
  Process_22/RConn4 -- Process_11/LConn9
  Process_22/RConn5 -- Process_14/LConn6
  Process_22/RConn6 -- Process_16/LConn12
  Process_22/RConn7 -- Process_22/LConn9
  Process_22/RConn8 -- Process_23/LConn11
  Process_22/RConn9 -- Process_25/LConn7
  Process_22/RConn10 -- Process_26/LConn9
  Process_22/RConn11 -- Process_30/LConn13
  Process_22/RConn12 -- Process_31/LConn6
  Process_22/RConn13 -- Process_33/LConn9
  Process_22/RConn14 -- Process_35/LConn7
  Process_22/RConn15 -- Process_38/LConn10
  Process_22/RConn16 -- Process_40/LConn10
  Process_22/RConn17 -- Process_41/LConn12
  Process_22/RConn18 -- Process_45/LConn8
  Process_22/RConn19 -- Process_47/LConn8
  Process_22/RConn20 -- Process_49/LConn7
  Process_22/RConn21 -- Process_53/LConn10
  Process_22/RConn22 -- Process_55/LConn9
  Process_22/RConn23 -- Process_58/LConn11
  Process_22/RConn24 -- Process_59/LConn12
  Process_22/RConn25 -- Process_64/LConn7
  Process_22/RConn26 -- Process_66/LConn9
  Process_22/RConn27 -- Process_67/LConn6
  Process_22/RConn28 -- Process_69/LConn9
  Process_22/RConn29 -- Process_73/LConn6
  Process_22/RConn30 -- Process_75/LConn9
  Process_22/RConn31 -- Process_76/LConn8
  Process_22/RConn32 -- Process_77/LConn9
  Process_22/RConn33 -- Process_78/LConn4
  Process_22/RConn34 -- Process_79/LConn11
  Process_22/RConn35 -- Process_84/LConn5
  Process_22/RConn36 -- Process_85/LConn6
  Process_22/RConn37 -- Process_87/LConn6
  Process_22/RConn38 -- Process_90/LConn10
  Process_22/RConn39 -- Process_91/LConn10
  Process_22/RConn40 -- Process_93/LConn11
  Process_22/RConn41 -- Process_95/LConn7
  Process_22/RConn42 -- Process_99/LConn15
  Process_23/RConn1 -- Process_8/LConn9
  Process_23/RConn2 -- Process_9/LConn11
  Process_23/RConn3 -- Process_10/LConn8
  Process_23/RConn4 -- Process_11/LConn10
  Process_23/RConn5 -- Process_12/LConn6
  Process_23/RConn6 -- Process_18/LConn10
  Process_23/RConn7 -- Process_19/LConn7
  Process_23/RConn8 -- Process_21/LConn8
  Process_23/RConn9 -- Process_32/LConn7
  Process_23/RConn10 -- Process_33/LConn10
  Process_23/RConn11 -- Process_35/LConn8
  Process_23/RConn12 -- Process_36/LConn9
  Process_23/RConn13 -- Process_37/LConn9
  Process_23/RConn14 -- Process_41/LConn13
  Process_23/RConn15 -- Process_42/LConn10
  Process_23/RConn16 -- Process_43/LConn11
  Process_23/RConn17 -- Process_45/LConn9
  Process_23/RConn18 -- Process_49/LConn8
  Process_23/RConn19 -- Process_52/LConn8
  Process_23/RConn20 -- Process_55/LConn10
  Process_23/RConn21 -- Process_56/LConn10
  Process_23/RConn22 -- Process_57/LConn8
  Process_23/RConn23 -- Process_61/LConn11
  Process_23/RConn24 -- Process_62/LConn9
  Process_23/RConn25 -- Process_69/LConn10
  Process_23/RConn26 -- Process_75/LConn10
  Process_23/RConn27 -- Process_78/LConn5
  Process_23/RConn28 -- Process_81/LConn9
  Process_23/RConn29 -- Process_84/LConn6
  Process_23/RConn30 -- Process_85/LConn7
  Process_23/RConn31 -- Process_87/LConn7
  Process_23/RConn32 -- Process_88/LConn8
  Process_23/RConn33 -- Process_92/LConn8
  Process_23/RConn34 -- Process_93/LConn12
  Process_23/RConn35 -- Process_100/LConn8
  Process_24/RConn1 -- Process_2/LConn8
  Process_24/RConn2 -- Process_4/LConn9
  Process_24/RConn3 -- Process_6/LConn13
  Process_24/RConn4 -- Process_7/LConn9
  Process_24/RConn5 -- Process_8/LConn10
  Process_24/RConn6 -- Process_10/LConn9
  Process_24/RConn7 -- Process_11/LConn11
  Process_24/RConn8 -- Process_13/LConn8
  Process_24/RConn9 -- Process_16/LConn13
  Process_24/RConn10 -- Process_23/LConn12
  Process_24/RConn11 -- Process_24/LConn6
  Process_24/RConn12 -- Process_32/LConn8
  Process_24/RConn13 -- Process_34/LConn8
  Process_24/RConn14 -- Process_37/LConn10
  Process_24/RConn15 -- Process_41/LConn14
  Process_24/RConn16 -- Process_45/LConn10
  Process_24/RConn17 -- Process_46/LConn10
  Process_24/RConn18 -- Process_49/LConn9
  Process_24/RConn19 -- Process_50/LConn12
  Process_24/RConn20 -- Process_51/LConn8
  Process_24/RConn21 -- Process_55/LConn11
  Process_24/RConn22 -- Process_60/LConn9
  Process_24/RConn23 -- Process_63/LConn6
  Process_24/RConn24 -- Process_65/LConn8
  Process_24/RConn25 -- Process_73/LConn7
  Process_24/RConn26 -- Process_76/LConn9
  Process_24/RConn27 -- Process_82/LConn12
  Process_24/RConn28 -- Process_85/LConn8
  Process_24/RConn29 -- Process_86/LConn8
  Process_24/RConn30 -- Process_88/LConn9
  Process_24/RConn31 -- Process_89/LConn9
  Process_24/RConn32 -- Process_90/LConn11
  Process_24/RConn33 -- Process_96/LConn8
  Process_24/RConn34 -- Process_97/LConn8
  Process_24/RConn35 -- Process_99/LConn16
  Process_25/RConn1 -- Process_1/LConn8
  Process_25/RConn2 -- Process_6/LConn14
  Process_25/RConn3 -- Process_11/LConn12
  Process_25/RConn4 -- Process_13/LConn9
  Process_25/RConn5 -- Process_17/LConn10
  Process_25/RConn6 -- Process_26/LConn10
  Process_25/RConn7 -- Process_30/LConn14
  Process_25/RConn8 -- Process_32/LConn9
  Process_25/RConn9 -- Process_33/LConn11
  Process_25/RConn10 -- Process_35/LConn9
  Process_25/RConn11 -- Process_37/LConn11
  Process_25/RConn12 -- Process_38/LConn11
  Process_25/RConn13 -- Process_40/LConn11
  Process_25/RConn14 -- Process_44/LConn9
  Process_25/RConn15 -- Process_47/LConn9
  Process_25/RConn16 -- Process_48/LConn8
  Process_25/RConn17 -- Process_49/LConn10
  Process_25/RConn18 -- Process_50/LConn13
  Process_25/RConn19 -- Process_51/LConn9
  Process_25/RConn20 -- Process_52/LConn9
  Process_25/RConn21 -- Process_55/LConn12
  Process_25/RConn22 -- Process_57/LConn9
  Process_25/RConn23 -- Process_62/LConn10
  Process_25/RConn24 -- Process_63/LConn7
  Process_25/RConn25 -- Process_68/LConn10
  Process_25/RConn26 -- Process_69/LConn11
  Process_25/RConn27 -- Process_72/LConn8
  Process_25/RConn28 -- Process_73/LConn8
  Process_25/RConn29 -- Process_74/LConn10
  Process_25/RConn30 -- Process_78/LConn6
  Process_25/RConn31 -- Process_79/LConn12
  Process_25/RConn32 -- Process_80/LConn9
  Process_25/RConn33 -- Process_81/LConn10
  Process_25/RConn34 -- Process_85/LConn9
  Process_25/RConn35 -- Process_86/LConn9
  Process_25/RConn36 -- Process_87/LConn8
  Process_25/RConn37 -- Process_89/LConn10
  Process_25/RConn38 -- Process_95/LConn8
  Process_25/RConn39 -- Process_96/LConn9
  Process_25/RConn40 -- Process_100/LConn9
  Process_26/RConn1 -- Process_1/LConn9
  Process_26/RConn2 -- Process_4/LConn10
  Process_26/RConn3 -- Process_6/LConn15
  Process_26/RConn4 -- Process_8/LConn11
  Process_26/RConn5 -- Process_11/LConn13
  Process_26/RConn6 -- Process_12/LConn7
  Process_26/RConn7 -- Process_13/LConn10
  Process_26/RConn8 -- Process_17/LConn11
  Process_26/RConn9 -- Process_23/LConn13
  Process_26/RConn10 -- Process_28/LConn8
  Process_26/RConn11 -- Process_29/LConn9
  Process_26/RConn12 -- Process_35/LConn10
  Process_26/RConn13 -- Process_36/LConn10
  Process_26/RConn14 -- Process_37/LConn12
  Process_26/RConn15 -- Process_39/LConn6
  Process_26/RConn16 -- Process_40/LConn12
  Process_26/RConn17 -- Process_46/LConn11
  Process_26/RConn18 -- Process_53/LConn11
  Process_26/RConn19 -- Process_55/LConn13
  Process_26/RConn20 -- Process_56/LConn11
  Process_26/RConn21 -- Process_58/LConn12
  Process_26/RConn22 -- Process_59/LConn13
  Process_26/RConn23 -- Process_60/LConn10
  Process_26/RConn24 -- Process_63/LConn8
  Process_26/RConn25 -- Process_64/LConn8
  Process_26/RConn26 -- Process_65/LConn9
  Process_26/RConn27 -- Process_69/LConn12
  Process_26/RConn28 -- Process_70/LConn8
  Process_26/RConn29 -- Process_77/LConn10
  Process_26/RConn30 -- Process_78/LConn7
  Process_26/RConn31 -- Process_80/LConn10
  Process_26/RConn32 -- Process_81/LConn11
  Process_26/RConn33 -- Process_85/LConn10
  Process_26/RConn34 -- Process_86/LConn10
  Process_26/RConn35 -- Process_87/LConn9
  Process_26/RConn36 -- Process_89/LConn11
  Process_26/RConn37 -- Process_91/LConn11
  Process_26/RConn38 -- Process_92/LConn9
  Process_26/RConn39 -- Process_97/LConn9
  Process_27/RConn1 -- Process_1/LConn10
  Process_27/RConn2 -- Process_3/LConn8
  Process_27/RConn3 -- Process_4/LConn11
  Process_27/RConn4 -- Process_5/LConn7
  Process_27/RConn5 -- Process_7/LConn10
  Process_27/RConn6 -- Process_8/LConn12
  Process_27/RConn7 -- Process_14/LConn7
  Process_27/RConn8 -- Process_16/LConn14
  Process_27/RConn9 -- Process_20/LConn5
  Process_27/RConn10 -- Process_22/LConn10
  Process_27/RConn11 -- Process_23/LConn14
  Process_27/RConn12 -- Process_25/LConn8
  Process_27/RConn13 -- Process_27/LConn8
  Process_27/RConn14 -- Process_32/LConn10
  Process_27/RConn15 -- Process_33/LConn12
  Process_27/RConn16 -- Process_40/LConn13
  Process_27/RConn17 -- Process_42/LConn11
  Process_27/RConn18 -- Process_44/LConn10
  Process_27/RConn19 -- Process_45/LConn11
  Process_27/RConn20 -- Process_46/LConn12
  Process_27/RConn21 -- Process_47/LConn10
  Process_27/RConn22 -- Process_50/LConn14
  Process_27/RConn23 -- Process_52/LConn10
  Process_27/RConn24 -- Process_53/LConn12
  Process_27/RConn25 -- Process_54/LConn6
  Process_27/RConn26 -- Process_56/LConn12
  Process_27/RConn27 -- Process_58/LConn13
  Process_27/RConn28 -- Process_59/LConn14
  Process_27/RConn29 -- Process_60/LConn11
  Process_27/RConn30 -- Process_63/LConn9
  Process_27/RConn31 -- Process_64/LConn9
  Process_27/RConn32 -- Process_67/LConn7
  Process_27/RConn33 -- Process_73/LConn9
  Process_27/RConn34 -- Process_75/LConn11
  Process_27/RConn35 -- Process_76/LConn10
  Process_27/RConn36 -- Process_83/LConn16
  Process_27/RConn37 -- Process_84/LConn7
  Process_27/RConn38 -- Process_85/LConn11
  Process_27/RConn39 -- Process_91/LConn12
  Process_27/RConn40 -- Process_95/LConn9
  Process_27/RConn41 -- Process_96/LConn10
  Process_27/RConn42 -- Process_98/LConn13
  Process_28/RConn1 -- Process_5/LConn8
  Process_28/RConn2 -- Process_7/LConn11
  Process_28/RConn3 -- Process_9/LConn12
  Process_28/RConn4 -- Process_11/LConn14
  Process_28/RConn5 -- Process_12/LConn8
  Process_28/RConn6 -- Process_13/LConn11
  Process_28/RConn7 -- Process_14/LConn8
  Process_28/RConn8 -- Process_17/LConn12
  Process_28/RConn9 -- Process_18/LConn11
  Process_28/RConn10 -- Process_20/LConn6
  Process_28/RConn11 -- Process_24/LConn7
  Process_28/RConn12 -- Process_26/LConn11
  Process_28/RConn13 -- Process_35/LConn11
  Process_28/RConn14 -- Process_36/LConn11
  Process_28/RConn15 -- Process_46/LConn13
  Process_28/RConn16 -- Process_53/LConn13
  Process_28/RConn17 -- Process_57/LConn10
  Process_28/RConn18 -- Process_59/LConn15
  Process_28/RConn19 -- Process_64/LConn10
  Process_28/RConn20 -- Process_65/LConn10
  Process_28/RConn21 -- Process_71/LConn11
  Process_28/RConn22 -- Process_74/LConn11
  Process_28/RConn23 -- Process_76/LConn11
  Process_28/RConn24 -- Process_84/LConn8
  Process_28/RConn25 -- Process_93/LConn13
  Process_28/RConn26 -- Process_96/LConn11
  Process_28/RConn27 -- Process_98/LConn14
  Process_28/RConn28 -- Process_99/LConn17
  Process_29/RConn1 -- Process_2/LConn9
  Process_29/RConn2 -- Process_4/LConn12
  Process_29/RConn3 -- Process_5/LConn9
  Process_29/RConn4 -- Process_8/LConn13
  Process_29/RConn5 -- Process_9/LConn13
  Process_29/RConn6 -- Process_12/LConn9
  Process_29/RConn7 -- Process_14/LConn9
  Process_29/RConn8 -- Process_17/LConn13
  Process_29/RConn9 -- Process_18/LConn12
  Process_29/RConn10 -- Process_25/LConn9
  Process_29/RConn11 -- Process_26/LConn12
  Process_29/RConn12 -- Process_35/LConn12
  Process_29/RConn13 -- Process_39/LConn7
  Process_29/RConn14 -- Process_41/LConn15
  Process_29/RConn15 -- Process_42/LConn12
  Process_29/RConn16 -- Process_44/LConn11
  Process_29/RConn17 -- Process_45/LConn12
  Process_29/RConn18 -- Process_46/LConn14
  Process_29/RConn19 -- Process_47/LConn11
  Process_29/RConn20 -- Process_48/LConn9
  Process_29/RConn21 -- Process_54/LConn7
  Process_29/RConn22 -- Process_55/LConn14
  Process_29/RConn23 -- Process_56/LConn13
  Process_29/RConn24 -- Process_61/LConn12
  Process_29/RConn25 -- Process_65/LConn11
  Process_29/RConn26 -- Process_68/LConn11
  Process_29/RConn27 -- Process_75/LConn12
  Process_29/RConn28 -- Process_76/LConn12
  Process_29/RConn29 -- Process_79/LConn13
  Process_29/RConn30 -- Process_84/LConn9
  Process_29/RConn31 -- Process_85/LConn12
  Process_29/RConn32 -- Process_88/LConn10
  Process_29/RConn33 -- Process_90/LConn12
  Process_29/RConn34 -- Process_94/LConn8
  Process_29/RConn35 -- Process_99/LConn18
  Process_29/RConn36 -- Process_100/LConn10
  Process_30/RConn1 -- Process_4/LConn13
  Process_30/RConn2 -- Process_9/LConn14
  Process_30/RConn3 -- Process_11/LConn15
  Process_30/RConn4 -- Process_14/LConn10
  Process_30/RConn5 -- Process_15/LConn9
  Process_30/RConn6 -- Process_16/LConn15
  Process_30/RConn7 -- Process_19/LConn8
  Process_30/RConn8 -- Process_22/LConn11
  Process_30/RConn9 -- Process_25/LConn10
  Process_30/RConn10 -- Process_27/LConn9
  Process_30/RConn11 -- Process_28/LConn9
  Process_30/RConn12 -- Process_31/LConn7
  Process_30/RConn13 -- Process_33/LConn13
  Process_30/RConn14 -- Process_34/LConn9
  Process_30/RConn15 -- Process_37/LConn13
  Process_30/RConn16 -- Process_41/LConn16
  Process_30/RConn17 -- Process_43/LConn12
  Process_30/RConn18 -- Process_45/LConn13
  Process_30/RConn19 -- Process_47/LConn12
  Process_30/RConn20 -- Process_50/LConn15
  Process_30/RConn21 -- Process_51/LConn10
  Process_30/RConn22 -- Process_53/LConn14
  Process_30/RConn23 -- Process_54/LConn8
  Process_30/RConn24 -- Process_55/LConn15
  Process_30/RConn25 -- Process_63/LConn10
  Process_30/RConn26 -- Process_70/LConn9
  Process_30/RConn27 -- Process_75/LConn13
  Process_30/RConn28 -- Process_78/LConn8
  Process_30/RConn29 -- Process_79/LConn14
  Process_30/RConn30 -- Process_80/LConn11
  Process_30/RConn31 -- Process_82/LConn13
  Process_30/RConn32 -- Process_85/LConn13
  Process_30/RConn33 -- Process_86/LConn11
  Process_30/RConn34 -- Process_92/LConn10
  Process_30/RConn35 -- Process_94/LConn9
  Process_30/RConn36 -- Process_96/LConn12
  Process_30/RConn37 -- Process_99/LConn19
  Process_31/RConn1 -- Process_1/LConn11
  Process_31/RConn2 -- Process_4/LConn14
  Process_31/RConn3 -- Process_9/LConn15
  Process_31/RConn4 -- Process_10/LConn10
  Process_31/RConn5 -- Process_12/LConn10
  Process_31/RConn6 -- Process_15/LConn10
  Process_31/RConn7 -- Process_18/LConn13
  Process_31/RConn8 -- Process_19/LConn9
  Process_31/RConn9 -- Process_23/LConn15
  Process_31/RConn10 -- Process_26/LConn13
  Process_31/RConn11 -- Process_38/LConn12
  Process_31/RConn12 -- Process_40/LConn14
  Process_31/RConn13 -- Process_42/LConn13
  Process_31/RConn14 -- Process_44/LConn12
  Process_31/RConn15 -- Process_45/LConn14
  Process_31/RConn16 -- Process_48/LConn10
  Process_31/RConn17 -- Process_49/LConn11
  Process_31/RConn18 -- Process_51/LConn11
  Process_31/RConn19 -- Process_56/LConn14
  Process_31/RConn20 -- Process_65/LConn12
  Process_31/RConn21 -- Process_67/LConn8
  Process_31/RConn22 -- Process_77/LConn11
  Process_31/RConn23 -- Process_79/LConn15
  Process_31/RConn24 -- Process_81/LConn12
  Process_31/RConn25 -- Process_94/LConn10
  Process_31/RConn26 -- Process_97/LConn10
  Process_31/RConn27 -- Process_100/LConn11
  Process_32/RConn1 -- Process_8/LConn14
  Process_32/RConn2 -- Process_9/LConn16
  Process_32/RConn3 -- Process_12/LConn11
  Process_32/RConn4 -- Process_13/LConn12
  Process_32/RConn5 -- Process_17/LConn14
  Process_32/RConn6 -- Process_20/LConn7
  Process_32/RConn7 -- Process_25/LConn11
  Process_32/RConn8 -- Process_26/LConn14
  Process_32/RConn9 -- Process_28/LConn10
  Process_32/RConn10 -- Process_31/LConn8
  Process_32/RConn11 -- Process_33/LConn14
  Process_32/RConn12 -- Process_34/LConn10
  Process_32/RConn13 -- Process_37/LConn14
  Process_32/RConn14 -- Process_38/LConn13
  Process_32/RConn15 -- Process_40/LConn15
  Process_32/RConn16 -- Process_41/LConn17
  Process_32/RConn17 -- Process_42/LConn14
  Process_32/RConn18 -- Process_43/LConn13
  Process_32/RConn19 -- Process_45/LConn15
  Process_32/RConn20 -- Process_47/LConn13
  Process_32/RConn21 -- Process_48/LConn11
  Process_32/RConn22 -- Process_51/LConn12
  Process_32/RConn23 -- Process_52/LConn11
  Process_32/RConn24 -- Process_55/LConn16
  Process_32/RConn25 -- Process_58/LConn14
  Process_32/RConn26 -- Process_63/LConn11
  Process_32/RConn27 -- Process_69/LConn13
  Process_32/RConn28 -- Process_71/LConn12
  Process_32/RConn29 -- Process_73/LConn10
  Process_32/RConn30 -- Process_74/LConn12
  Process_32/RConn31 -- Process_76/LConn13
  Process_32/RConn32 -- Process_77/LConn12
  Process_32/RConn33 -- Process_85/LConn14
  Process_32/RConn34 -- Process_87/LConn10
  Process_32/RConn35 -- Process_89/LConn12
  Process_32/RConn36 -- Process_93/LConn14
  Process_32/RConn37 -- Process_96/LConn13
  Process_33/RConn1 -- Process_2/LConn10
  Process_33/RConn2 -- Process_3/LConn9
  Process_33/RConn3 -- Process_6/LConn16
  Process_33/RConn4 -- Process_9/LConn17
  Process_33/RConn5 -- Process_12/LConn12
  Process_33/RConn6 -- Process_13/LConn13
  Process_33/RConn7 -- Process_14/LConn11
  Process_33/RConn8 -- Process_16/LConn16
  Process_33/RConn9 -- Process_18/LConn14
  Process_33/RConn10 -- Process_19/LConn10
  Process_33/RConn11 -- Process_21/LConn9
  Process_33/RConn12 -- Process_23/LConn16
  Process_33/RConn13 -- Process_24/LConn8
  Process_33/RConn14 -- Process_26/LConn15
  Process_33/RConn15 -- Process_27/LConn10
  Process_33/RConn16 -- Process_40/LConn16
  Process_33/RConn17 -- Process_42/LConn15
  Process_33/RConn18 -- Process_44/LConn13
  Process_33/RConn19 -- Process_49/LConn12
  Process_33/RConn20 -- Process_51/LConn13
  Process_33/RConn21 -- Process_53/LConn15
  Process_33/RConn22 -- Process_54/LConn9
  Process_33/RConn23 -- Process_55/LConn17
  Process_33/RConn24 -- Process_57/LConn11
  Process_33/RConn25 -- Process_59/LConn16
  Process_33/RConn26 -- Process_62/LConn11
  Process_33/RConn27 -- Process_64/LConn11
  Process_33/RConn28 -- Process_65/LConn13
  Process_33/RConn29 -- Process_66/LConn10
  Process_33/RConn30 -- Process_67/LConn9
  Process_33/RConn31 -- Process_69/LConn14
  Process_33/RConn32 -- Process_71/LConn13
  Process_33/RConn33 -- Process_72/LConn9
  Process_33/RConn34 -- Process_77/LConn13
  Process_33/RConn35 -- Process_83/LConn17
  Process_33/RConn36 -- Process_84/LConn10
  Process_33/RConn37 -- Process_89/LConn13
  Process_33/RConn38 -- Process_90/LConn13
  Process_33/RConn39 -- Process_92/LConn11
  Process_33/RConn40 -- Process_93/LConn15
  Process_33/RConn41 -- Process_98/LConn15
  Process_34/RConn1 -- Process_1/LConn12
  Process_34/RConn2 -- Process_7/LConn12
  Process_34/RConn3 -- Process_10/LConn11
  Process_34/RConn4 -- Process_11/LConn16
  Process_34/RConn5 -- Process_13/LConn14
  Process_34/RConn6 -- Process_19/LConn11
  Process_34/RConn7 -- Process_25/LConn12
  Process_34/RConn8 -- Process_29/LConn10
  Process_34/RConn9 -- Process_31/LConn9
  Process_34/RConn10 -- Process_36/LConn12
  Process_34/RConn11 -- Process_37/LConn15
  Process_34/RConn12 -- Process_40/LConn17
  Process_34/RConn13 -- Process_43/LConn14
  Process_34/RConn14 -- Process_44/LConn14
  Process_34/RConn15 -- Process_46/LConn15
  Process_34/RConn16 -- Process_47/LConn14
  Process_34/RConn17 -- Process_49/LConn13
  Process_34/RConn18 -- Process_50/LConn16
  Process_34/RConn19 -- Process_52/LConn12
  Process_34/RConn20 -- Process_55/LConn18
  Process_34/RConn21 -- Process_59/LConn17
  Process_34/RConn22 -- Process_60/LConn12
  Process_34/RConn23 -- Process_62/LConn12
  Process_34/RConn24 -- Process_64/LConn12
  Process_34/RConn25 -- Process_65/LConn14
  Process_34/RConn26 -- Process_66/LConn11
  Process_34/RConn27 -- Process_67/LConn10
  Process_34/RConn28 -- Process_68/LConn12
  Process_34/RConn29 -- Process_69/LConn15
  Process_34/RConn30 -- Process_71/LConn14
  Process_34/RConn31 -- Process_72/LConn10
  Process_34/RConn32 -- Process_73/LConn11
  Process_34/RConn33 -- Process_75/LConn14
  Process_34/RConn34 -- Process_78/LConn9
  Process_34/RConn35 -- Process_88/LConn11
  Process_34/RConn36 -- Process_89/LConn14
  Process_34/RConn37 -- Process_90/LConn14
  Process_34/RConn38 -- Process_93/LConn16
  Process_34/RConn39 -- Process_97/LConn11
  Process_35/RConn1 -- Process_6/LConn17
  Process_35/RConn2 -- Process_7/LConn13
  Process_35/RConn3 -- Process_9/LConn18
  Process_35/RConn4 -- Process_14/LConn12
  Process_35/RConn5 -- Process_18/LConn15
  Process_35/RConn6 -- Process_21/LConn10
  Process_35/RConn7 -- Process_23/LConn17
  Process_35/RConn8 -- Process_25/LConn13
  Process_35/RConn9 -- Process_29/LConn11
  Process_35/RConn10 -- Process_34/LConn11
  Process_35/RConn11 -- Process_38/LConn14
  Process_35/RConn12 -- Process_41/LConn18
  Process_35/RConn13 -- Process_45/LConn16
  Process_35/RConn14 -- Process_47/LConn15
  Process_35/RConn15 -- Process_50/LConn17
  Process_35/RConn16 -- Process_51/LConn14
  Process_35/RConn17 -- Process_53/LConn16
  Process_35/RConn18 -- Process_55/LConn19
  Process_35/RConn19 -- Process_56/LConn15
  Process_35/RConn20 -- Process_57/LConn12
  Process_35/RConn21 -- Process_61/LConn13
  Process_35/RConn22 -- Process_62/LConn13
  Process_35/RConn23 -- Process_64/LConn13
  Process_35/RConn24 -- Process_65/LConn15
  Process_35/RConn25 -- Process_66/LConn12
  Process_35/RConn26 -- Process_68/LConn13
  Process_35/RConn27 -- Process_71/LConn15
  Process_35/RConn28 -- Process_73/LConn12
  Process_35/RConn29 -- Process_77/LConn14
  Process_35/RConn30 -- Process_82/LConn14
  Process_35/RConn31 -- Process_84/LConn11
  Process_35/RConn32 -- Process_85/LConn15
  Process_35/RConn33 -- Process_88/LConn12
  Process_35/RConn34 -- Process_89/LConn15
  Process_35/RConn35 -- Process_96/LConn14
  Process_35/RConn36 -- Process_98/LConn16
  Process_35/RConn37 -- Process_99/LConn20
  Process_36/RConn1 -- Process_2/LConn11
  Process_36/RConn2 -- Process_3/LConn10
  Process_36/RConn3 -- Process_5/LConn10
  Process_36/RConn4 -- Process_9/LConn19
  Process_36/RConn5 -- Process_11/LConn17
  Process_36/RConn6 -- Process_13/LConn15
  Process_36/RConn7 -- Process_16/LConn17
  Process_36/RConn8 -- Process_17/LConn15
  Process_36/RConn9 -- Process_18/LConn16
  Process_36/RConn10 -- Process_23/LConn18
  Process_36/RConn11 -- Process_24/LConn9
  Process_36/RConn12 -- Process_26/LConn16
  Process_36/RConn13 -- Process_31/LConn10
  Process_36/RConn14 -- Process_32/LConn11
  Process_36/RConn15 -- Process_38/LConn15
  Process_36/RConn16 -- Process_44/LConn15
  Process_36/RConn17 -- Process_52/LConn13
  Process_36/RConn18 -- Process_54/LConn10
  Process_36/RConn19 -- Process_56/LConn16
  Process_36/RConn20 -- Process_57/LConn13
  Process_36/RConn21 -- Process_61/LConn14
  Process_36/RConn22 -- Process_62/LConn14
  Process_36/RConn23 -- Process_63/LConn12
  Process_36/RConn24 -- Process_67/LConn11
  Process_36/RConn25 -- Process_68/LConn14
  Process_36/RConn26 -- Process_71/LConn16
  Process_36/RConn27 -- Process_75/LConn15
  Process_36/RConn28 -- Process_77/LConn15
  Process_36/RConn29 -- Process_79/LConn16
  Process_36/RConn30 -- Process_83/LConn18
  Process_36/RConn31 -- Process_84/LConn12
  Process_36/RConn32 -- Process_88/LConn13
  Process_36/RConn33 -- Process_95/LConn10
  Process_36/RConn34 -- Process_96/LConn15
  Process_36/RConn35 -- Process_98/LConn17
  Process_37/RConn1 -- Process_3/LConn11
  Process_37/RConn2 -- Process_8/LConn15
  Process_37/RConn3 -- Process_11/LConn18
  Process_37/RConn4 -- Process_12/LConn13
  Process_37/RConn5 -- Process_13/LConn16
  Process_37/RConn6 -- Process_14/LConn13
  Process_37/RConn7 -- Process_15/LConn11
  Process_37/RConn8 -- Process_16/LConn18
  Process_37/RConn9 -- Process_21/LConn11
  Process_37/RConn10 -- Process_25/LConn14
  Process_37/RConn11 -- Process_26/LConn17
  Process_37/RConn12 -- Process_27/LConn11
  Process_37/RConn13 -- Process_29/LConn12
  Process_37/RConn14 -- Process_36/LConn13
  Process_37/RConn15 -- Process_42/LConn16
  Process_37/RConn16 -- Process_44/LConn16
  Process_37/RConn17 -- Process_51/LConn15
  Process_37/RConn18 -- Process_54/LConn11
  Process_37/RConn19 -- Process_55/LConn20
  Process_37/RConn20 -- Process_60/LConn13
  Process_37/RConn21 -- Process_62/LConn15
  Process_37/RConn22 -- Process_63/LConn13
  Process_37/RConn23 -- Process_69/LConn16
  Process_37/RConn24 -- Process_71/LConn17
  Process_37/RConn25 -- Process_75/LConn16
  Process_37/RConn26 -- Process_78/LConn10
  Process_37/RConn27 -- Process_79/LConn17
  Process_37/RConn28 -- Process_81/LConn13
  Process_37/RConn29 -- Process_86/LConn12
  Process_37/RConn30 -- Process_87/LConn11
  Process_37/RConn31 -- Process_91/LConn13
  Process_37/RConn32 -- Process_94/LConn11
  Process_37/RConn33 -- Process_96/LConn16
  Process_37/RConn34 -- Process_97/LConn12
  Process_38/RConn1 -- Process_1/LConn13
  Process_38/RConn2 -- Process_3/LConn12
  Process_38/RConn3 -- Process_4/LConn15
  Process_38/RConn4 -- Process_5/LConn11
  Process_38/RConn5 -- Process_6/LConn18
  Process_38/RConn6 -- Process_12/LConn14
  Process_38/RConn7 -- Process_13/LConn17
  Process_38/RConn8 -- Process_14/LConn14
  Process_38/RConn9 -- Process_18/LConn17
  Process_38/RConn10 -- Process_24/LConn10
  Process_38/RConn11 -- Process_25/LConn15
  Process_38/RConn12 -- Process_26/LConn18
  Process_38/RConn13 -- Process_28/LConn11
  Process_38/RConn14 -- Process_36/LConn14
  Process_38/RConn15 -- Process_39/LConn8
  Process_38/RConn16 -- Process_41/LConn19
  Process_38/RConn17 -- Process_42/LConn17
  Process_38/RConn18 -- Process_47/LConn16
  Process_38/RConn19 -- Process_48/LConn12
  Process_38/RConn20 -- Process_51/LConn16
  Process_38/RConn21 -- Process_55/LConn21
  Process_38/RConn22 -- Process_56/LConn17
  Process_38/RConn23 -- Process_57/LConn14
  Process_38/RConn24 -- Process_58/LConn15
  Process_38/RConn25 -- Process_59/LConn18
  Process_38/RConn26 -- Process_61/LConn15
  Process_38/RConn27 -- Process_62/LConn16
  Process_38/RConn28 -- Process_65/LConn16
  Process_38/RConn29 -- Process_67/LConn12
  Process_38/RConn30 -- Process_68/LConn15
  Process_38/RConn31 -- Process_69/LConn17
  Process_38/RConn32 -- Process_79/LConn18
  Process_38/RConn33 -- Process_91/LConn14
  Process_38/RConn34 -- Process_92/LConn12
  Process_38/RConn35 -- Process_93/LConn17
  Process_38/RConn36 -- Process_98/LConn18
  Process_38/RConn37 -- Process_99/LConn21
  Process_39/RConn1 -- Process_2/LConn12
  Process_39/RConn2 -- Process_6/LConn19
  Process_39/RConn3 -- Process_7/LConn14
  Process_39/RConn4 -- Process_9/LConn20
  Process_39/RConn5 -- Process_11/LConn19
  Process_39/RConn6 -- Process_13/LConn18
  Process_39/RConn7 -- Process_14/LConn15
  Process_39/RConn8 -- Process_17/LConn16
  Process_39/RConn9 -- Process_18/LConn18
  Process_39/RConn10 -- Process_19/LConn12
  Process_39/RConn11 -- Process_23/LConn19
  Process_39/RConn12 -- Process_24/LConn11
  Process_39/RConn13 -- Process_26/LConn19
  Process_39/RConn14 -- Process_27/LConn12
  Process_39/RConn15 -- Process_29/LConn13
  Process_39/RConn16 -- Process_30/LConn15
  Process_39/RConn17 -- Process_32/LConn12
  Process_39/RConn18 -- Process_35/LConn13
  Process_39/RConn19 -- Process_41/LConn20
  Process_39/RConn20 -- Process_47/LConn17
  Process_39/RConn21 -- Process_48/LConn13
  Process_39/RConn22 -- Process_49/LConn14
  Process_39/RConn23 -- Process_50/LConn18
  Process_39/RConn24 -- Process_54/LConn12
  Process_39/RConn25 -- Process_58/LConn16
  Process_39/RConn26 -- Process_59/LConn19
  Process_39/RConn27 -- Process_60/LConn14
  Process_39/RConn28 -- Process_63/LConn14
  Process_39/RConn29 -- Process_70/LConn10
  Process_39/RConn30 -- Process_72/LConn11
  Process_39/RConn31 -- Process_81/LConn14
  Process_39/RConn32 -- Process_83/LConn19
  Process_39/RConn33 -- Process_84/LConn13
  Process_39/RConn34 -- Process_87/LConn12
  Process_39/RConn35 -- Process_93/LConn18
  Process_39/RConn36 -- Process_96/LConn17
  Process_39/RConn37 -- Process_99/LConn22
  Process_40/RConn1 -- Process_1/LConn14
  Process_40/RConn2 -- Process_5/LConn12
  Process_40/RConn3 -- Process_7/LConn15
  Process_40/RConn4 -- Process_9/LConn21
  Process_40/RConn5 -- Process_10/LConn12
  Process_40/RConn6 -- Process_12/LConn15
  Process_40/RConn7 -- Process_14/LConn16
  Process_40/RConn8 -- Process_15/LConn12
  Process_40/RConn9 -- Process_20/LConn8
  Process_40/RConn10 -- Process_22/LConn12
  Process_40/RConn11 -- Process_23/LConn20
  Process_40/RConn12 -- Process_27/LConn13
  Process_40/RConn13 -- Process_32/LConn13
  Process_40/RConn14 -- Process_33/LConn15
  Process_40/RConn15 -- Process_34/LConn12
  Process_40/RConn16 -- Process_36/LConn15
  Process_40/RConn17 -- Process_38/LConn16
  Process_40/RConn18 -- Process_39/LConn9
  Process_40/RConn19 -- Process_40/LConn18
  Process_40/RConn20 -- Process_41/LConn21
  Process_40/RConn21 -- Process_42/LConn18
  Process_40/RConn22 -- Process_43/LConn15
  Process_40/RConn23 -- Process_44/LConn17
  Process_40/RConn24 -- Process_50/LConn19
  Process_40/RConn25 -- Process_52/LConn14
  Process_40/RConn26 -- Process_56/LConn18
  Process_40/RConn27 -- Process_57/LConn15
  Process_40/RConn28 -- Process_60/LConn15
  Process_40/RConn29 -- Process_63/LConn15
  Process_40/RConn30 -- Process_64/LConn14
  Process_40/RConn31 -- Process_66/LConn13
  Process_40/RConn32 -- Process_67/LConn13
  Process_40/RConn33 -- Process_68/LConn16
  Process_40/RConn34 -- Process_70/LConn11
  Process_40/RConn35 -- Process_72/LConn12
  Process_40/RConn36 -- Process_75/LConn17
  Process_40/RConn37 -- Process_77/LConn16
  Process_40/RConn38 -- Process_83/LConn20
  Process_40/RConn39 -- Process_84/LConn14
  Process_40/RConn40 -- Process_87/LConn13
  Process_40/RConn41 -- Process_91/LConn15
  Process_40/RConn42 -- Process_95/LConn11
  Process_40/RConn43 -- Process_99/LConn23
  Process_40/RConn44 -- Process_100/LConn12
  Process_41/RConn1 -- Process_1/LConn15
  Process_41/RConn2 -- Process_2/LConn13
  Process_41/RConn3 -- Process_5/LConn13
  Process_41/RConn4 -- Process_7/LConn16
  Process_41/RConn5 -- Process_8/LConn16
  Process_41/RConn6 -- Process_11/LConn20
  Process_41/RConn7 -- Process_13/LConn19
  Process_41/RConn8 -- Process_14/LConn17
  Process_41/RConn9 -- Process_15/LConn13
  Process_41/RConn10 -- Process_16/LConn19
  Process_41/RConn11 -- Process_17/LConn17
  Process_41/RConn12 -- Process_19/LConn13
  Process_41/RConn13 -- Process_23/LConn21
  Process_41/RConn14 -- Process_24/LConn12
  Process_41/RConn15 -- Process_25/LConn16
  Process_41/RConn16 -- Process_27/LConn14
  Process_41/RConn17 -- Process_28/LConn12
  Process_41/RConn18 -- Process_29/LConn14
  Process_41/RConn19 -- Process_30/LConn16
  Process_41/RConn20 -- Process_32/LConn14
  Process_41/RConn21 -- Process_34/LConn13
  Process_41/RConn22 -- Process_35/LConn14
  Process_41/RConn23 -- Process_39/LConn10
  Process_41/RConn24 -- Process_41/LConn22
  Process_41/RConn25 -- Process_42/LConn19
  Process_41/RConn26 -- Process_46/LConn16
  Process_41/RConn27 -- Process_47/LConn18
  Process_41/RConn28 -- Process_51/LConn17
  Process_41/RConn29 -- Process_52/LConn15
  Process_41/RConn30 -- Process_53/LConn17
  Process_41/RConn31 -- Process_57/LConn16
  Process_41/RConn32 -- Process_58/LConn17
  Process_41/RConn33 -- Process_59/LConn20
  Process_41/RConn34 -- Process_61/LConn16
  Process_41/RConn35 -- Process_63/LConn16
  Process_41/RConn36 -- Process_64/LConn15
  Process_41/RConn37 -- Process_69/LConn18
  Process_41/RConn38 -- Process_70/LConn12
  Process_41/RConn39 -- Process_72/LConn13
  Process_41/RConn40 -- Process_73/LConn13
  Process_41/RConn41 -- Process_77/LConn17
  Process_41/RConn42 -- Process_82/LConn15
  Process_41/RConn43 -- Process_83/LConn21
  Process_41/RConn44 -- Process_87/LConn14
  Process_41/RConn45 -- Process_89/LConn16
  Process_41/RConn46 -- Process_92/LConn13
  Process_42/RConn1 -- Process_3/LConn13
  Process_42/RConn2 -- Process_4/LConn16
  Process_42/RConn3 -- Process_5/LConn14
  Process_42/RConn4 -- Process_7/LConn17
  Process_42/RConn5 -- Process_8/LConn17
  Process_42/RConn6 -- Process_9/LConn22
  Process_42/RConn7 -- Process_20/LConn9
  Process_42/RConn8 -- Process_22/LConn13
  Process_42/RConn9 -- Process_23/LConn22
  Process_42/RConn10 -- Process_26/LConn20
  Process_42/RConn11 -- Process_27/LConn15
  Process_42/RConn12 -- Process_28/LConn13
  Process_42/RConn13 -- Process_33/LConn16
  Process_42/RConn14 -- Process_35/LConn15
  Process_42/RConn15 -- Process_37/LConn16
  Process_42/RConn16 -- Process_43/LConn16
  Process_42/RConn17 -- Process_45/LConn17
  Process_42/RConn18 -- Process_47/LConn19
  Process_42/RConn19 -- Process_55/LConn22
  Process_42/RConn20 -- Process_56/LConn19
  Process_42/RConn21 -- Process_63/LConn17
  Process_42/RConn22 -- Process_64/LConn16
  Process_42/RConn23 -- Process_69/LConn19
  Process_42/RConn24 -- Process_71/LConn18
  Process_42/RConn25 -- Process_73/LConn14
  Process_42/RConn26 -- Process_74/LConn13
  Process_42/RConn27 -- Process_80/LConn12
  Process_42/RConn28 -- Process_82/LConn16
  Process_42/RConn29 -- Process_85/LConn16
  Process_42/RConn30 -- Process_90/LConn15
  Process_42/RConn31 -- Process_92/LConn14
  Process_42/RConn32 -- Process_93/LConn19
  Process_42/RConn33 -- Process_94/LConn12
  Process_42/RConn34 -- Process_96/LConn18
  Process_43/RConn1 -- Process_7/LConn18
  Process_43/RConn2 -- Process_9/LConn23
  Process_43/RConn3 -- Process_11/LConn21
  Process_43/RConn4 -- Process_12/LConn16
  Process_43/RConn5 -- Process_16/LConn20
  Process_43/RConn6 -- Process_18/LConn19
  Process_43/RConn7 -- Process_22/LConn14
  Process_43/RConn8 -- Process_27/LConn16
  Process_43/RConn9 -- Process_28/LConn14
  Process_43/RConn10 -- Process_29/LConn15
  Process_43/RConn11 -- Process_32/LConn15
  Process_43/RConn12 -- Process_33/LConn17
  Process_43/RConn13 -- Process_34/LConn14
  Process_43/RConn14 -- Process_38/LConn17
  Process_43/RConn15 -- Process_40/LConn19
  Process_43/RConn16 -- Process_41/LConn23
  Process_43/RConn17 -- Process_43/LConn17
  Process_43/RConn18 -- Process_44/LConn18
  Process_43/RConn19 -- Process_48/LConn14
  Process_43/RConn20 -- Process_51/LConn18
  Process_43/RConn21 -- Process_52/LConn16
  Process_43/RConn22 -- Process_53/LConn18
  Process_43/RConn23 -- Process_55/LConn23
  Process_43/RConn24 -- Process_56/LConn20
  Process_43/RConn25 -- Process_57/LConn17
  Process_43/RConn26 -- Process_61/LConn17
  Process_43/RConn27 -- Process_62/LConn17
  Process_43/RConn28 -- Process_65/LConn17
  Process_43/RConn29 -- Process_73/LConn15
  Process_43/RConn30 -- Process_75/LConn18
  Process_43/RConn31 -- Process_78/LConn11
  Process_43/RConn32 -- Process_79/LConn19
  Process_43/RConn33 -- Process_81/LConn15
  Process_43/RConn34 -- Process_83/LConn22
  Process_43/RConn35 -- Process_86/LConn13
  Process_43/RConn36 -- Process_87/LConn15
  Process_43/RConn37 -- Process_89/LConn17
  Process_43/RConn38 -- Process_90/LConn16
  Process_43/RConn39 -- Process_92/LConn15
  Process_43/RConn40 -- Process_94/LConn13
  Process_43/RConn41 -- Process_96/LConn19
  Process_44/RConn1 -- Process_2/LConn14
  Process_44/RConn2 -- Process_3/LConn14
  Process_44/RConn3 -- Process_4/LConn17
  Process_44/RConn4 -- Process_7/LConn19
  Process_44/RConn5 -- Process_10/LConn13
  Process_44/RConn6 -- Process_14/LConn18
  Process_44/RConn7 -- Process_15/LConn14
  Process_44/RConn8 -- Process_16/LConn21
  Process_44/RConn9 -- Process_18/LConn20
  Process_44/RConn10 -- Process_21/LConn12
  Process_44/RConn11 -- Process_22/LConn15
  Process_44/RConn12 -- Process_24/LConn13
  Process_44/RConn13 -- Process_25/LConn17
  Process_44/RConn14 -- Process_27/LConn17
  Process_44/RConn15 -- Process_30/LConn17
  Process_44/RConn16 -- Process_34/LConn15
  Process_44/RConn17 -- Process_40/LConn20
  Process_44/RConn18 -- Process_43/LConn18
  Process_44/RConn19 -- Process_48/LConn15
  Process_44/RConn20 -- Process_49/LConn15
  Process_44/RConn21 -- Process_50/LConn20
  Process_44/RConn22 -- Process_52/LConn17
  Process_44/RConn23 -- Process_54/LConn13
  Process_44/RConn24 -- Process_56/LConn21
  Process_44/RConn25 -- Process_63/LConn18
  Process_44/RConn26 -- Process_64/LConn17
  Process_44/RConn27 -- Process_66/LConn14
  Process_44/RConn28 -- Process_67/LConn14
  Process_44/RConn29 -- Process_69/LConn20
  Process_44/RConn30 -- Process_73/LConn16
  Process_44/RConn31 -- Process_74/LConn14
  Process_44/RConn32 -- Process_75/LConn19
  Process_44/RConn33 -- Process_76/LConn14
  Process_44/RConn34 -- Process_82/LConn17
  Process_44/RConn35 -- Process_86/LConn14
  Process_44/RConn36 -- Process_87/LConn16
  Process_44/RConn37 -- Process_88/LConn14
  Process_44/RConn38 -- Process_89/LConn18
  Process_44/RConn39 -- Process_90/LConn17
  Process_44/RConn40 -- Process_91/LConn16
  Process_44/RConn41 -- Process_92/LConn16
  Process_44/RConn42 -- Process_94/LConn14
  Process_44/RConn43 -- Process_96/LConn20
  Process_44/RConn44 -- Process_97/LConn13
  Process_44/RConn45 -- Process_98/LConn19
  Process_45/RConn1 -- Process_1/LConn16
  Process_45/RConn2 -- Process_3/LConn15
  Process_45/RConn3 -- Process_4/LConn18
  Process_45/RConn4 -- Process_7/LConn20
  Process_45/RConn5 -- Process_10/LConn14
  Process_45/RConn6 -- Process_13/LConn20
  Process_45/RConn7 -- Process_19/LConn14
  Process_45/RConn8 -- Process_23/LConn23
  Process_45/RConn9 -- Process_27/LConn18
  Process_45/RConn10 -- Process_31/LConn11
  Process_45/RConn11 -- Process_33/LConn18
  Process_45/RConn12 -- Process_34/LConn16
  Process_45/RConn13 -- Process_38/LConn18
  Process_45/RConn14 -- Process_41/LConn24
  Process_45/RConn15 -- Process_43/LConn19
  Process_45/RConn16 -- Process_46/LConn17
  Process_45/RConn17 -- Process_49/LConn16
  Process_45/RConn18 -- Process_52/LConn18
  Process_45/RConn19 -- Process_58/LConn18
  Process_45/RConn20 -- Process_60/LConn16
  Process_45/RConn21 -- Process_68/LConn17
  Process_45/RConn22 -- Process_71/LConn19
  Process_45/RConn23 -- Process_76/LConn15
  Process_45/RConn24 -- Process_84/LConn15
  Process_45/RConn25 -- Process_85/LConn17
  Process_45/RConn26 -- Process_87/LConn17
  Process_45/RConn27 -- Process_89/LConn19
  Process_45/RConn28 -- Process_90/LConn18
  Process_45/RConn29 -- Process_91/LConn17
  Process_45/RConn30 -- Process_92/LConn17
  Process_45/RConn31 -- Process_94/LConn15
  Process_45/RConn32 -- Process_95/LConn12
  Process_45/RConn33 -- Process_96/LConn21
  Process_45/RConn34 -- Process_98/LConn20
  Process_45/RConn35 -- Process_100/LConn13
  Process_46/RConn1 -- Process_6/LConn20
  Process_46/RConn2 -- Process_9/LConn24
  Process_46/RConn3 -- Process_10/LConn15
  Process_46/RConn4 -- Process_14/LConn19
  Process_46/RConn5 -- Process_15/LConn15
  Process_46/RConn6 -- Process_18/LConn21
  Process_46/RConn7 -- Process_20/LConn10
  Process_46/RConn8 -- Process_21/LConn13
  Process_46/RConn9 -- Process_22/LConn16
  Process_46/RConn10 -- Process_34/LConn17
  Process_46/RConn11 -- Process_37/LConn17
  Process_46/RConn12 -- Process_40/LConn21
  Process_46/RConn13 -- Process_43/LConn20
  Process_46/RConn14 -- Process_44/LConn19
  Process_46/RConn15 -- Process_47/LConn20
  Process_46/RConn16 -- Process_48/LConn16
  Process_46/RConn17 -- Process_49/LConn17
  Process_46/RConn18 -- Process_50/LConn21
  Process_46/RConn19 -- Process_53/LConn19
  Process_46/RConn20 -- Process_54/LConn14
  Process_46/RConn21 -- Process_57/LConn18
  Process_46/RConn22 -- Process_58/LConn19
  Process_46/RConn23 -- Process_59/LConn21
  Process_46/RConn24 -- Process_61/LConn18
  Process_46/RConn25 -- Process_63/LConn19
  Process_46/RConn26 -- Process_66/LConn15
  Process_46/RConn27 -- Process_68/LConn18
  Process_46/RConn28 -- Process_69/LConn21
  Process_46/RConn29 -- Process_71/LConn20
  Process_46/RConn30 -- Process_73/LConn17
  Process_46/RConn31 -- Process_75/LConn20
  Process_46/RConn32 -- Process_76/LConn16
  Process_46/RConn33 -- Process_77/LConn18
  Process_46/RConn34 -- Process_78/LConn12
  Process_46/RConn35 -- Process_83/LConn23
  Process_46/RConn36 -- Process_89/LConn20
  Process_46/RConn37 -- Process_91/LConn18
  Process_46/RConn38 -- Process_92/LConn18
  Process_46/RConn39 -- Process_94/LConn16
  Process_46/RConn40 -- Process_99/LConn24
  Process_47/RConn1 -- Process_4/LConn19
  Process_47/RConn2 -- Process_7/LConn21
  Process_47/RConn3 -- Process_18/LConn22
  Process_47/RConn4 -- Process_23/LConn24
  Process_47/RConn5 -- Process_26/LConn21
  Process_47/RConn6 -- Process_32/LConn16
  Process_47/RConn7 -- Process_33/LConn19
  Process_47/RConn8 -- Process_34/LConn18
  Process_47/RConn9 -- Process_35/LConn16
  Process_47/RConn10 -- Process_37/LConn18
  Process_47/RConn11 -- Process_38/LConn19
  Process_47/RConn12 -- Process_43/LConn21
  Process_47/RConn13 -- Process_45/LConn18
  Process_47/RConn14 -- Process_46/LConn18
  Process_47/RConn15 -- Process_47/LConn21
  Process_47/RConn16 -- Process_48/LConn17
  Process_47/RConn17 -- Process_50/LConn22
  Process_47/RConn18 -- Process_51/LConn19
  Process_47/RConn19 -- Process_55/LConn24
  Process_47/RConn20 -- Process_59/LConn22
  Process_47/RConn21 -- Process_63/LConn20
  Process_47/RConn22 -- Process_69/LConn22
  Process_47/RConn23 -- Process_73/LConn18
  Process_47/RConn24 -- Process_78/LConn13
  Process_47/RConn25 -- Process_81/LConn16
  Process_47/RConn26 -- Process_82/LConn18
  Process_47/RConn27 -- Process_88/LConn15
  Process_47/RConn28 -- Process_90/LConn19
  Process_47/RConn29 -- Process_91/LConn19
  Process_47/RConn30 -- Process_96/LConn22
  Process_47/RConn31 -- Process_97/LConn14
  Process_47/RConn32 -- Process_98/LConn21
  Process_47/RConn33 -- Process_99/LConn25
  Process_48/RConn1 -- Process_2/LConn15
  Process_48/RConn2 -- Process_4/LConn20
  Process_48/RConn3 -- Process_6/LConn21
  Process_48/RConn4 -- Process_7/LConn22
  Process_48/RConn5 -- Process_8/LConn18
  Process_48/RConn6 -- Process_11/LConn22
  Process_48/RConn7 -- Process_12/LConn17
  Process_48/RConn8 -- Process_13/LConn21
  Process_48/RConn9 -- Process_14/LConn20
  Process_48/RConn10 -- Process_15/LConn16
  Process_48/RConn11 -- Process_17/LConn18
  Process_48/RConn12 -- Process_23/LConn25
  Process_48/RConn13 -- Process_24/LConn14
  Process_48/RConn14 -- Process_26/LConn22
  Process_48/RConn15 -- Process_30/LConn18
  Process_48/RConn16 -- Process_33/LConn20
  Process_48/RConn17 -- Process_34/LConn19
  Process_48/RConn18 -- Process_36/LConn16
  Process_48/RConn19 -- Process_38/LConn20
  Process_48/RConn20 -- Process_39/LConn11
  Process_48/RConn21 -- Process_41/LConn25
  Process_48/RConn22 -- Process_48/LConn18
  Process_48/RConn23 -- Process_49/LConn18
  Process_48/RConn24 -- Process_51/LConn20
  Process_48/RConn25 -- Process_53/LConn20
  Process_48/RConn26 -- Process_64/LConn18
  Process_48/RConn27 -- Process_75/LConn21
  Process_48/RConn28 -- Process_79/LConn20
  Process_48/RConn29 -- Process_81/LConn17
  Process_48/RConn30 -- Process_82/LConn19
  Process_48/RConn31 -- Process_85/LConn18
  Process_48/RConn32 -- Process_86/LConn15
  Process_48/RConn33 -- Process_92/LConn19
  Process_48/RConn34 -- Process_94/LConn17
  Process_48/RConn35 -- Process_95/LConn13
  Process_48/RConn36 -- Process_99/LConn26
  Process_49/RConn1 -- Process_3/LConn16
  Process_49/RConn2 -- Process_9/LConn25
  Process_49/RConn3 -- Process_10/LConn16
  Process_49/RConn4 -- Process_11/LConn23
  Process_49/RConn5 -- Process_13/LConn22
  Process_49/RConn6 -- Process_14/LConn21
  Process_49/RConn7 -- Process_16/LConn22
  Process_49/RConn8 -- Process_17/LConn19
  Process_49/RConn9 -- Process_20/LConn11
  Process_49/RConn10 -- Process_23/LConn26
  Process_49/RConn11 -- Process_24/LConn15
  Process_49/RConn12 -- Process_25/LConn18
  Process_49/RConn13 -- Process_26/LConn23
  Process_49/RConn14 -- Process_29/LConn16
  Process_49/RConn15 -- Process_32/LConn17
  Process_49/RConn16 -- Process_35/LConn17
  Process_49/RConn17 -- Process_40/LConn22
  Process_49/RConn18 -- Process_41/LConn26
  Process_49/RConn19 -- Process_46/LConn19
  Process_49/RConn20 -- Process_48/LConn19
  Process_49/RConn21 -- Process_50/LConn23
  Process_49/RConn22 -- Process_52/LConn19
  Process_49/RConn23 -- Process_55/LConn25
  Process_49/RConn24 -- Process_59/LConn23
  Process_49/RConn25 -- Process_60/LConn17
  Process_49/RConn26 -- Process_64/LConn19
  Process_49/RConn27 -- Process_65/LConn18
  Process_49/RConn28 -- Process_70/LConn13
  Process_49/RConn29 -- Process_71/LConn21
  Process_49/RConn30 -- Process_72/LConn14
  Process_49/RConn31 -- Process_76/LConn17
  Process_49/RConn32 -- Process_78/LConn14
  Process_49/RConn33 -- Process_80/LConn13
  Process_49/RConn34 -- Process_81/LConn18
  Process_49/RConn35 -- Process_83/LConn24
  Process_49/RConn36 -- Process_86/LConn16
  Process_49/RConn37 -- Process_89/LConn21
  Process_49/RConn38 -- Process_91/LConn20
  Process_49/RConn39 -- Process_95/LConn14
  Process_50/RConn1 -- Process_7/LConn23
  Process_50/RConn2 -- Process_8/LConn19
  Process_50/RConn3 -- Process_14/LConn22
  Process_50/RConn4 -- Process_18/LConn23
  Process_50/RConn5 -- Process_19/LConn15
  Process_50/RConn6 -- Process_21/LConn14
  Process_50/RConn7 -- Process_25/LConn19
  Process_50/RConn8 -- Process_27/LConn19
  Process_50/RConn9 -- Process_34/LConn20
  Process_50/RConn10 -- Process_39/LConn12
  Process_50/RConn11 -- Process_40/LConn23
  Process_50/RConn12 -- Process_41/LConn27
  Process_50/RConn13 -- Process_44/LConn20
  Process_50/RConn14 -- Process_48/LConn20
  Process_50/RConn15 -- Process_49/LConn19
  Process_50/RConn16 -- Process_51/LConn21
  Process_50/RConn17 -- Process_52/LConn20
  Process_50/RConn18 -- Process_54/LConn15
  Process_50/RConn19 -- Process_55/LConn26
  Process_50/RConn20 -- Process_56/LConn22
  Process_50/RConn21 -- Process_59/LConn24
  Process_50/RConn22 -- Process_61/LConn19
  Process_50/RConn23 -- Process_62/LConn18
  Process_50/RConn24 -- Process_63/LConn21
  Process_50/RConn25 -- Process_65/LConn19
  Process_50/RConn26 -- Process_67/LConn15
  Process_50/RConn27 -- Process_68/LConn19
  Process_50/RConn28 -- Process_69/LConn23
  Process_50/RConn29 -- Process_70/LConn14
  Process_50/RConn30 -- Process_76/LConn18
  Process_50/RConn31 -- Process_78/LConn15
  Process_50/RConn32 -- Process_79/LConn21
  Process_50/RConn33 -- Process_81/LConn19
  Process_50/RConn34 -- Process_85/LConn19
  Process_50/RConn35 -- Process_86/LConn17
  Process_50/RConn36 -- Process_88/LConn16
  Process_50/RConn37 -- Process_94/LConn18
  Process_50/RConn38 -- Process_97/LConn15
  Process_50/RConn39 -- Process_98/LConn22
  Process_50/RConn40 -- Process_99/LConn27
  Process_51/RConn1 -- Process_3/LConn17
  Process_51/RConn2 -- Process_6/LConn22
  Process_51/RConn3 -- Process_7/LConn24
  Process_51/RConn4 -- Process_9/LConn26
  Process_51/RConn5 -- Process_11/LConn24
  Process_51/RConn6 -- Process_19/LConn16
  Process_51/RConn7 -- Process_22/LConn17
  Process_51/RConn8 -- Process_26/LConn24
  Process_51/RConn9 -- Process_27/LConn20
  Process_51/RConn10 -- Process_29/LConn17
  Process_51/RConn11 -- Process_30/LConn19
  Process_51/RConn12 -- Process_31/LConn12
  Process_51/RConn13 -- Process_32/LConn18
  Process_51/RConn14 -- Process_34/LConn21
  Process_51/RConn15 -- Process_40/LConn24
  Process_51/RConn16 -- Process_41/LConn28
  Process_51/RConn17 -- Process_54/LConn16
  Process_51/RConn18 -- Process_55/LConn27
  Process_51/RConn19 -- Process_56/LConn23
  Process_51/RConn20 -- Process_58/LConn20
  Process_51/RConn21 -- Process_65/LConn20
  Process_51/RConn22 -- Process_66/LConn16
  Process_51/RConn23 -- Process_67/LConn16
  Process_51/RConn24 -- Process_73/LConn19
  Process_51/RConn25 -- Process_74/LConn15
  Process_51/RConn26 -- Process_76/LConn19
  Process_51/RConn27 -- Process_77/LConn19
  Process_51/RConn28 -- Process_80/LConn14
  Process_51/RConn29 -- Process_82/LConn20
  Process_51/RConn30 -- Process_83/LConn25
  Process_51/RConn31 -- Process_84/LConn16
  Process_51/RConn32 -- Process_87/LConn18
  Process_51/RConn33 -- Process_89/LConn22
  Process_51/RConn34 -- Process_92/LConn20
  Process_51/RConn35 -- Process_94/LConn19
  Process_51/RConn36 -- Process_96/LConn23
  Process_51/RConn37 -- Process_99/LConn28
  Process_52/RConn1 -- Process_1/LConn17
  Process_52/RConn2 -- Process_7/LConn25
  Process_52/RConn3 -- Process_11/LConn25
  Process_52/RConn4 -- Process_12/LConn18
  Process_52/RConn5 -- Process_18/LConn24
  Process_52/RConn6 -- Process_19/LConn17
  Process_52/RConn7 -- Process_22/LConn18
  Process_52/RConn8 -- Process_23/LConn27
  Process_52/RConn9 -- Process_24/LConn16
  Process_52/RConn10 -- Process_27/LConn21
  Process_52/RConn11 -- Process_33/LConn21
  Process_52/RConn12 -- Process_37/LConn19
  Process_52/RConn13 -- Process_40/LConn25
  Process_52/RConn14 -- Process_43/LConn22
  Process_52/RConn15 -- Process_44/LConn21
  Process_52/RConn16 -- Process_45/LConn19
  Process_52/RConn17 -- Process_47/LConn22
  Process_52/RConn18 -- Process_50/LConn24
  Process_52/RConn19 -- Process_54/LConn17
  Process_52/RConn20 -- Process_56/LConn24
  Process_52/RConn21 -- Process_58/LConn21
  Process_52/RConn22 -- Process_59/LConn25
  Process_52/RConn23 -- Process_60/LConn18
  Process_52/RConn24 -- Process_61/LConn20
  Process_52/RConn25 -- Process_63/LConn22
  Process_52/RConn26 -- Process_73/LConn20
  Process_52/RConn27 -- Process_76/LConn20
  Process_52/RConn28 -- Process_84/LConn17
  Process_52/RConn29 -- Process_87/LConn19
  Process_52/RConn30 -- Process_89/LConn23
  Process_52/RConn31 -- Process_90/LConn20
  Process_52/RConn32 -- Process_93/LConn20
  Process_52/RConn33 -- Process_95/LConn15
  Process_52/RConn34 -- Process_96/LConn24
  Process_53/RConn1 -- Process_1/LConn18
  Process_53/RConn2 -- Process_2/LConn16
  Process_53/RConn3 -- Process_5/LConn15
  Process_53/RConn4 -- Process_7/LConn26
  Process_53/RConn5 -- Process_14/LConn23
  Process_53/RConn6 -- Process_17/LConn20
  Process_53/RConn7 -- Process_20/LConn12
  Process_53/RConn8 -- Process_27/LConn22
  Process_53/RConn9 -- Process_28/LConn15
  Process_53/RConn10 -- Process_31/LConn13
  Process_53/RConn11 -- Process_34/LConn22
  Process_53/RConn12 -- Process_35/LConn18
  Process_53/RConn13 -- Process_39/LConn13
  Process_53/RConn14 -- Process_40/LConn26
  Process_53/RConn15 -- Process_41/LConn29
  Process_53/RConn16 -- Process_42/LConn20
  Process_53/RConn17 -- Process_44/LConn22
  Process_53/RConn18 -- Process_46/LConn20
  Process_53/RConn19 -- Process_48/LConn21
  Process_53/RConn20 -- Process_51/LConn22
  Process_53/RConn21 -- Process_54/LConn18
  Process_53/RConn22 -- Process_55/LConn28
  Process_53/RConn23 -- Process_59/LConn26
  Process_53/RConn24 -- Process_60/LConn19
  Process_53/RConn25 -- Process_62/LConn19
  Process_53/RConn26 -- Process_63/LConn23
  Process_53/RConn27 -- Process_64/LConn20
  Process_53/RConn28 -- Process_66/LConn17
  Process_53/RConn29 -- Process_75/LConn22
  Process_53/RConn30 -- Process_79/LConn22
  Process_53/RConn31 -- Process_85/LConn20
  Process_53/RConn32 -- Process_86/LConn18
  Process_53/RConn33 -- Process_87/LConn20
  Process_53/RConn34 -- Process_89/LConn24
  Process_53/RConn35 -- Process_90/LConn21
  Process_53/RConn36 -- Process_92/LConn21
  Process_53/RConn37 -- Process_95/LConn16
  Process_53/RConn38 -- Process_98/LConn23
  Process_54/RConn1 -- Process_1/LConn19
  Process_54/RConn2 -- Process_5/LConn16
  Process_54/RConn3 -- Process_6/LConn23
  Process_54/RConn4 -- Process_11/LConn26
  Process_54/RConn5 -- Process_12/LConn19
  Process_54/RConn6 -- Process_13/LConn23
  Process_54/RConn7 -- Process_16/LConn23
  Process_54/RConn8 -- Process_19/LConn18
  Process_54/RConn9 -- Process_21/LConn15
  Process_54/RConn10 -- Process_23/LConn28
  Process_54/RConn11 -- Process_25/LConn20
  Process_54/RConn12 -- Process_26/LConn25
  Process_54/RConn13 -- Process_31/LConn14
  Process_54/RConn14 -- Process_39/LConn14
  Process_54/RConn15 -- Process_40/LConn27
  Process_54/RConn16 -- Process_41/LConn30
  Process_54/RConn17 -- Process_42/LConn21
  Process_54/RConn18 -- Process_43/LConn23
  Process_54/RConn19 -- Process_47/LConn23
  Process_54/RConn20 -- Process_48/LConn22
  Process_54/RConn21 -- Process_50/LConn25
  Process_54/RConn22 -- Process_51/LConn23
  Process_54/RConn23 -- Process_54/LConn19
  Process_54/RConn24 -- Process_56/LConn25
  Process_54/RConn25 -- Process_59/LConn27
  Process_54/RConn26 -- Process_60/LConn20
  Process_54/RConn27 -- Process_61/LConn21
  Process_54/RConn28 -- Process_62/LConn20
  Process_54/RConn29 -- Process_63/LConn24
  Process_54/RConn30 -- Process_64/LConn21
  Process_54/RConn31 -- Process_67/LConn17
  Process_54/RConn32 -- Process_68/LConn20
  Process_54/RConn33 -- Process_70/LConn15
  Process_54/RConn34 -- Process_71/LConn22
  Process_54/RConn35 -- Process_73/LConn21
  Process_54/RConn36 -- Process_75/LConn23
  Process_54/RConn37 -- Process_77/LConn20
  Process_54/RConn38 -- Process_78/LConn16
  Process_54/RConn39 -- Process_81/LConn20
  Process_54/RConn40 -- Process_82/LConn21
  Process_54/RConn41 -- Process_84/LConn18
  Process_54/RConn42 -- Process_85/LConn21
  Process_54/RConn43 -- Process_86/LConn19
  Process_54/RConn44 -- Process_87/LConn21
  Process_54/RConn45 -- Process_88/LConn17
  Process_54/RConn46 -- Process_89/LConn25
  Process_54/RConn47 -- Process_92/LConn22
  Process_54/RConn48 -- Process_93/LConn21
  Process_54/RConn49 -- Process_95/LConn17
  Process_54/RConn50 -- Process_100/LConn14
  Process_55/RConn1 -- Process_2/LConn17
  Process_55/RConn2 -- Process_4/LConn21
  Process_55/RConn3 -- Process_8/LConn20
  Process_55/RConn4 -- Process_10/LConn17
  Process_55/RConn5 -- Process_15/LConn17
  Process_55/RConn6 -- Process_17/LConn21
  Process_55/RConn7 -- Process_19/LConn19
  Process_55/RConn8 -- Process_20/LConn13
  Process_55/RConn9 -- Process_22/LConn19
  Process_55/RConn10 -- Process_23/LConn29
  Process_55/RConn11 -- Process_25/LConn21
  Process_55/RConn12 -- Process_29/LConn18
  Process_55/RConn13 -- Process_31/LConn15
  Process_55/RConn14 -- Process_32/LConn19
  Process_55/RConn15 -- Process_33/LConn22
  Process_55/RConn16 -- Process_36/LConn17
  Process_55/RConn17 -- Process_38/LConn21
  Process_55/RConn18 -- Process_39/LConn15
  Process_55/RConn19 -- Process_40/LConn28
  Process_55/RConn20 -- Process_46/LConn21
  Process_55/RConn21 -- Process_47/LConn24
  Process_55/RConn22 -- Process_48/LConn23
  Process_55/RConn23 -- Process_51/LConn24
  Process_55/RConn24 -- Process_53/LConn21
  Process_55/RConn25 -- Process_54/LConn20
  Process_55/RConn26 -- Process_55/LConn29
  Process_55/RConn27 -- Process_58/LConn22
  Process_55/RConn28 -- Process_60/LConn21
  Process_55/RConn29 -- Process_61/LConn22
  Process_55/RConn30 -- Process_65/LConn21
  Process_55/RConn31 -- Process_66/LConn18
  Process_55/RConn32 -- Process_67/LConn18
  Process_55/RConn33 -- Process_68/LConn21
  Process_55/RConn34 -- Process_74/LConn16
  Process_55/RConn35 -- Process_76/LConn21
  Process_55/RConn36 -- Process_77/LConn21
  Process_55/RConn37 -- Process_78/LConn17
  Process_55/RConn38 -- Process_79/LConn23
  Process_55/RConn39 -- Process_81/LConn21
  Process_55/RConn40 -- Process_82/LConn22
  Process_55/RConn41 -- Process_84/LConn19
  Process_55/RConn42 -- Process_87/LConn22
  Process_55/RConn43 -- Process_90/LConn22
  Process_55/RConn44 -- Process_91/LConn21
  Process_55/RConn45 -- Process_100/LConn15
  Process_56/RConn1 -- Process_2/LConn18
  Process_56/RConn2 -- Process_3/LConn18
  Process_56/RConn3 -- Process_5/LConn17
  Process_56/RConn4 -- Process_6/LConn24
  Process_56/RConn5 -- Process_7/LConn27
  Process_56/RConn6 -- Process_9/LConn27
  Process_56/RConn7 -- Process_10/LConn18
  Process_56/RConn8 -- Process_11/LConn27
  Process_56/RConn9 -- Process_14/LConn24
  Process_56/RConn10 -- Process_17/LConn22
  Process_56/RConn11 -- Process_20/LConn14
  Process_56/RConn12 -- Process_27/LConn23
  Process_56/RConn13 -- Process_28/LConn16
  Process_56/RConn14 -- Process_34/LConn23
  Process_56/RConn15 -- Process_35/LConn19
  Process_56/RConn16 -- Process_41/LConn31
  Process_56/RConn17 -- Process_43/LConn24
  Process_56/RConn18 -- Process_44/LConn23
  Process_56/RConn19 -- Process_46/LConn22
  Process_56/RConn20 -- Process_49/LConn20
  Process_56/RConn21 -- Process_54/LConn21
  Process_56/RConn22 -- Process_55/LConn30
  Process_56/RConn23 -- Process_56/LConn26
  Process_56/RConn24 -- Process_58/LConn23
  Process_56/RConn25 -- Process_60/LConn22
  Process_56/RConn26 -- Process_61/LConn23
  Process_56/RConn27 -- Process_64/LConn22
  Process_56/RConn28 -- Process_65/LConn22
  Process_56/RConn29 -- Process_66/LConn19
  Process_56/RConn30 -- Process_71/LConn23
  Process_56/RConn31 -- Process_79/LConn24
  Process_56/RConn32 -- Process_80/LConn15
  Process_56/RConn33 -- Process_85/LConn22
  Process_56/RConn34 -- Process_87/LConn23
  Process_56/RConn35 -- Process_88/LConn18
  Process_56/RConn36 -- Process_91/LConn22
  Process_56/RConn37 -- Process_94/LConn20
  Process_56/RConn38 -- Process_100/LConn16
  Process_57/RConn1 -- Process_6/LConn25
  Process_57/RConn2 -- Process_8/LConn21
  Process_57/RConn3 -- Process_11/LConn28
  Process_57/RConn4 -- Process_13/LConn24
  Process_57/RConn5 -- Process_14/LConn25
  Process_57/RConn6 -- Process_16/LConn24
  Process_57/RConn7 -- Process_22/LConn20
  Process_57/RConn8 -- Process_24/LConn17
  Process_57/RConn9 -- Process_30/LConn20
  Process_57/RConn10 -- Process_34/LConn24
  Process_57/RConn11 -- Process_39/LConn16
  Process_57/RConn12 -- Process_40/LConn29
  Process_57/RConn13 -- Process_42/LConn22
  Process_57/RConn14 -- Process_45/LConn20
  Process_57/RConn15 -- Process_46/LConn23
  Process_57/RConn16 -- Process_51/LConn25
  Process_57/RConn17 -- Process_55/LConn31
  Process_57/RConn18 -- Process_56/LConn27
  Process_57/RConn19 -- Process_57/LConn19
  Process_57/RConn20 -- Process_63/LConn25
  Process_57/RConn21 -- Process_71/LConn24
  Process_57/RConn22 -- Process_73/LConn22
  Process_57/RConn23 -- Process_76/LConn22
  Process_57/RConn24 -- Process_77/LConn22
  Process_57/RConn25 -- Process_82/LConn23
  Process_57/RConn26 -- Process_83/LConn26
  Process_57/RConn27 -- Process_84/LConn20
  Process_57/RConn28 -- Process_89/LConn26
  Process_57/RConn29 -- Process_92/LConn23
  Process_57/RConn30 -- Process_99/LConn29
  Process_57/RConn31 -- Process_100/LConn17
  Process_58/RConn1 -- Process_3/LConn19
  Process_58/RConn2 -- Process_4/LConn22
  Process_58/RConn3 -- Process_6/LConn26
  Process_58/RConn4 -- Process_8/LConn22
  Process_58/RConn5 -- Process_16/LConn25
  Process_58/RConn6 -- Process_17/LConn23
  Process_58/RConn7 -- Process_19/LConn20
  Process_58/RConn8 -- Process_20/LConn15
  Process_58/RConn9 -- Process_22/LConn21
  Process_58/RConn10 -- Process_26/LConn26
  Process_58/RConn11 -- Process_27/LConn24
  Process_58/RConn12 -- Process_29/LConn19
  Process_58/RConn13 -- Process_30/LConn21
  Process_58/RConn14 -- Process_36/LConn18
  Process_58/RConn15 -- Process_37/LConn20
  Process_58/RConn16 -- Process_38/LConn22
  Process_58/RConn17 -- Process_39/LConn17
  Process_58/RConn18 -- Process_40/LConn30
  Process_58/RConn19 -- Process_41/LConn32
  Process_58/RConn20 -- Process_44/LConn24
  Process_58/RConn21 -- Process_45/LConn21
  Process_58/RConn22 -- Process_46/LConn24
  Process_58/RConn23 -- Process_48/LConn24
  Process_58/RConn24 -- Process_49/LConn21
  Process_58/RConn25 -- Process_50/LConn26
  Process_58/RConn26 -- Process_51/LConn26
  Process_58/RConn27 -- Process_54/LConn22
  Process_58/RConn28 -- Process_55/LConn32
  Process_58/RConn29 -- Process_56/LConn28
  Process_58/RConn30 -- Process_58/LConn24
  Process_58/RConn31 -- Process_62/LConn21
  Process_58/RConn32 -- Process_65/LConn23
  Process_58/RConn33 -- Process_66/LConn20
  Process_58/RConn34 -- Process_70/LConn16
  Process_58/RConn35 -- Process_71/LConn25
  Process_58/RConn36 -- Process_76/LConn23
  Process_58/RConn37 -- Process_86/LConn20
  Process_58/RConn38 -- Process_90/LConn23
  Process_58/RConn39 -- Process_93/LConn22
  Process_58/RConn40 -- Process_94/LConn21
  Process_58/RConn41 -- Process_98/LConn24
  Process_58/RConn42 -- Process_99/LConn30
  Process_59/RConn1 -- Process_3/LConn20
  Process_59/RConn2 -- Process_5/LConn18
  Process_59/RConn3 -- Process_10/LConn19
  Process_59/RConn4 -- Process_11/LConn29
  Process_59/RConn5 -- Process_12/LConn20
  Process_59/RConn6 -- Process_13/LConn25
  Process_59/RConn7 -- Process_24/LConn18
  Process_59/RConn8 -- Process_25/LConn22
  Process_59/RConn9 -- Process_27/LConn25
  Process_59/RConn10 -- Process_37/LConn21
  Process_59/RConn11 -- Process_38/LConn23
  Process_59/RConn12 -- Process_39/LConn18
  Process_59/RConn13 -- Process_41/LConn33
  Process_59/RConn14 -- Process_43/LConn25
  Process_59/RConn15 -- Process_45/LConn22
  Process_59/RConn16 -- Process_46/LConn25
  Process_59/RConn17 -- Process_48/LConn25
  Process_59/RConn18 -- Process_49/LConn22
  Process_59/RConn19 -- Process_50/LConn27
  Process_59/RConn20 -- Process_52/LConn21
  Process_59/RConn21 -- Process_54/LConn23
  Process_59/RConn22 -- Process_59/LConn28
  Process_59/RConn23 -- Process_61/LConn24
  Process_59/RConn24 -- Process_63/LConn26
  Process_59/RConn25 -- Process_66/LConn21
  Process_59/RConn26 -- Process_67/LConn19
  Process_59/RConn27 -- Process_70/LConn17
  Process_59/RConn28 -- Process_72/LConn15
  Process_59/RConn29 -- Process_73/LConn23
  Process_59/RConn30 -- Process_74/LConn17
  Process_59/RConn31 -- Process_75/LConn24
  Process_59/RConn32 -- Process_77/LConn23
  Process_59/RConn33 -- Process_78/LConn18
  Process_59/RConn34 -- Process_81/LConn22
  Process_59/RConn35 -- Process_83/LConn27
  Process_59/RConn36 -- Process_84/LConn21
  Process_59/RConn37 -- Process_85/LConn23
  Process_59/RConn38 -- Process_87/LConn24
  Process_59/RConn39 -- Process_88/LConn19
  Process_59/RConn40 -- Process_90/LConn24
  Process_59/RConn41 -- Process_93/LConn23
  Process_59/RConn42 -- Process_96/LConn25
  Process_59/RConn43 -- Process_100/LConn18
  Process_60/RConn1 -- Process_1/LConn20
  Process_60/RConn2 -- Process_6/LConn27
  Process_60/RConn3 -- Process_9/LConn28
  Process_60/RConn4 -- Process_10/LConn20
  Process_60/RConn5 -- Process_11/LConn30
  Process_60/RConn6 -- Process_12/LConn21
  Process_60/RConn7 -- Process_13/LConn26
  Process_60/RConn8 -- Process_17/LConn24
  Process_60/RConn9 -- Process_18/LConn25
  Process_60/RConn10 -- Process_19/LConn21
  Process_60/RConn11 -- Process_20/LConn16
  Process_60/RConn12 -- Process_23/LConn30
  Process_60/RConn13 -- Process_25/LConn23
  Process_60/RConn14 -- Process_28/LConn17
  Process_60/RConn15 -- Process_29/LConn20
  Process_60/RConn16 -- Process_32/LConn20
  Process_60/RConn17 -- Process_33/LConn23
  Process_60/RConn18 -- Process_34/LConn25
  Process_60/RConn19 -- Process_36/LConn19
  Process_60/RConn20 -- Process_38/LConn24
  Process_60/RConn21 -- Process_42/LConn23
  Process_60/RConn22 -- Process_45/LConn23
  Process_60/RConn23 -- Process_49/LConn23
  Process_60/RConn24 -- Process_51/LConn27
  Process_60/RConn25 -- Process_54/LConn24
  Process_60/RConn26 -- Process_58/LConn25
  Process_60/RConn27 -- Process_60/LConn23
  Process_60/RConn28 -- Process_61/LConn25
  Process_60/RConn29 -- Process_64/LConn23
  Process_60/RConn30 -- Process_69/LConn24
  Process_60/RConn31 -- Process_74/LConn18
  Process_60/RConn32 -- Process_78/LConn19
  Process_60/RConn33 -- Process_79/LConn25
  Process_60/RConn34 -- Process_80/LConn16
  Process_60/RConn35 -- Process_81/LConn23
  Process_60/RConn36 -- Process_85/LConn24
  Process_60/RConn37 -- Process_86/LConn21
  Process_60/RConn38 -- Process_91/LConn23
  Process_60/RConn39 -- Process_94/LConn22
  Process_60/RConn40 -- Process_100/LConn19
  Process_61/RConn1 -- Process_4/LConn23
  Process_61/RConn2 -- Process_6/LConn28
  Process_61/RConn3 -- Process_10/LConn21
  Process_61/RConn4 -- Process_11/LConn31
  Process_61/RConn5 -- Process_15/LConn18
  Process_61/RConn6 -- Process_17/LConn25
  Process_61/RConn7 -- Process_18/LConn26
  Process_61/RConn8 -- Process_19/LConn22
  Process_61/RConn9 -- Process_20/LConn17
  Process_61/RConn10 -- Process_26/LConn27
  Process_61/RConn11 -- Process_27/LConn26
  Process_61/RConn12 -- Process_29/LConn21
  Process_61/RConn13 -- Process_33/LConn24
  Process_61/RConn14 -- Process_35/LConn20
  Process_61/RConn15 -- Process_38/LConn25
  Process_61/RConn16 -- Process_39/LConn19
  Process_61/RConn17 -- Process_42/LConn24
  Process_61/RConn18 -- Process_43/LConn26
  Process_61/RConn19 -- Process_46/LConn26
  Process_61/RConn20 -- Process_47/LConn25
  Process_61/RConn21 -- Process_52/LConn22
  Process_61/RConn22 -- Process_53/LConn22
  Process_61/RConn23 -- Process_55/LConn33
  Process_61/RConn24 -- Process_61/LConn26
  Process_61/RConn25 -- Process_62/LConn22
  Process_61/RConn26 -- Process_63/LConn27
  Process_61/RConn27 -- Process_68/LConn22
  Process_61/RConn28 -- Process_70/LConn18
  Process_61/RConn29 -- Process_73/LConn24
  Process_61/RConn30 -- Process_74/LConn19
  Process_61/RConn31 -- Process_75/LConn25
  Process_61/RConn32 -- Process_76/LConn24
  Process_61/RConn33 -- Process_78/LConn20
  Process_61/RConn34 -- Process_79/LConn26
  Process_61/RConn35 -- Process_80/LConn17
  Process_61/RConn36 -- Process_81/LConn24
  Process_61/RConn37 -- Process_84/LConn22
  Process_61/RConn38 -- Process_86/LConn22
  Process_61/RConn39 -- Process_90/LConn25
  Process_61/RConn40 -- Process_91/LConn24
  Process_61/RConn41 -- Process_93/LConn24
  Process_61/RConn42 -- Process_94/LConn23
  Process_61/RConn43 -- Process_100/LConn20
  Process_62/RConn1 -- Process_2/LConn19
  Process_62/RConn2 -- Process_4/LConn24
  Process_62/RConn3 -- Process_8/LConn23
  Process_62/RConn4 -- Process_10/LConn22
  Process_62/RConn5 -- Process_11/LConn32
  Process_62/RConn6 -- Process_17/LConn26
  Process_62/RConn7 -- Process_20/LConn18
  Process_62/RConn8 -- Process_22/LConn22
  Process_62/RConn9 -- Process_28/LConn18
  Process_62/RConn10 -- Process_30/LConn22
  Process_62/RConn11 -- Process_32/LConn21
  Process_62/RConn12 -- Process_33/LConn25
  Process_62/RConn13 -- Process_34/LConn26
  Process_62/RConn14 -- Process_36/LConn20
  Process_62/RConn15 -- Process_44/LConn25
  Process_62/RConn16 -- Process_45/LConn24
  Process_62/RConn17 -- Process_49/LConn24
  Process_62/RConn18 -- Process_56/LConn29
  Process_62/RConn19 -- Process_59/LConn29
  Process_62/RConn20 -- Process_60/LConn24
  Process_62/RConn21 -- Process_63/LConn28
  Process_62/RConn22 -- Process_64/LConn24
  Process_62/RConn23 -- Process_65/LConn24
  Process_62/RConn24 -- Process_66/LConn22
  Process_62/RConn25 -- Process_70/LConn19
  Process_62/RConn26 -- Process_72/LConn16
  Process_62/RConn27 -- Process_74/LConn20
  Process_62/RConn28 -- Process_76/LConn25
  Process_62/RConn29 -- Process_77/LConn24
  Process_62/RConn30 -- Process_78/LConn21
  Process_62/RConn31 -- Process_83/LConn28
  Process_62/RConn32 -- Process_85/LConn25
  Process_62/RConn33 -- Process_86/LConn23
  Process_62/RConn34 -- Process_87/LConn25
  Process_62/RConn35 -- Process_90/LConn26
  Process_62/RConn36 -- Process_93/LConn25
  Process_62/RConn37 -- Process_94/LConn24
  Process_62/RConn38 -- Process_97/LConn16
  Process_62/RConn39 -- Process_99/LConn31
  Process_62/RConn40 -- Process_100/LConn21
  Process_63/RConn1 -- Process_3/LConn21
  Process_63/RConn2 -- Process_4/LConn25
  Process_63/RConn3 -- Process_6/LConn29
  Process_63/RConn4 -- Process_7/LConn28
  Process_63/RConn5 -- Process_9/LConn29
  Process_63/RConn6 -- Process_14/LConn26
  Process_63/RConn7 -- Process_15/LConn19
  Process_63/RConn8 -- Process_19/LConn23
  Process_63/RConn9 -- Process_20/LConn19
  Process_63/RConn10 -- Process_21/LConn16
  Process_63/RConn11 -- Process_24/LConn19
  Process_63/RConn12 -- Process_30/LConn23
  Process_63/RConn13 -- Process_31/LConn16
  Process_63/RConn14 -- Process_32/LConn22
  Process_63/RConn15 -- Process_35/LConn21
  Process_63/RConn16 -- Process_36/LConn21
  Process_63/RConn17 -- Process_38/LConn26
  Process_63/RConn18 -- Process_40/LConn31
  Process_63/RConn19 -- Process_44/LConn26
  Process_63/RConn20 -- Process_46/LConn27
  Process_63/RConn21 -- Process_50/LConn28
  Process_63/RConn22 -- Process_52/LConn23
  Process_63/RConn23 -- Process_54/LConn25
  Process_63/RConn24 -- Process_57/LConn20
  Process_63/RConn25 -- Process_59/LConn30
  Process_63/RConn26 -- Process_60/LConn25
  Process_63/RConn27 -- Process_61/LConn27
  Process_63/RConn28 -- Process_66/LConn23
  Process_63/RConn29 -- Process_67/LConn20
  Process_63/RConn30 -- Process_69/LConn25
  Process_63/RConn31 -- Process_70/LConn20
  Process_63/RConn32 -- Process_71/LConn26
  Process_63/RConn33 -- Process_75/LConn26
  Process_63/RConn34 -- Process_77/LConn25
  Process_63/RConn35 -- Process_79/LConn27
  Process_63/RConn36 -- Process_84/LConn23
  Process_63/RConn37 -- Process_85/LConn26
  Process_63/RConn38 -- Process_88/LConn20
  Process_63/RConn39 -- Process_91/LConn25
  Process_63/RConn40 -- Process_98/LConn25
  Process_63/RConn41 -- Process_100/LConn22
  Process_64/RConn1 -- Process_1/LConn21
  Process_64/RConn2 -- Process_6/LConn30
  Process_64/RConn3 -- Process_7/LConn29
  Process_64/RConn4 -- Process_8/LConn24
  Process_64/RConn5 -- Process_10/LConn23
  Process_64/RConn6 -- Process_15/LConn20
  Process_64/RConn7 -- Process_17/LConn27
  Process_64/RConn8 -- Process_18/LConn27
  Process_64/RConn9 -- Process_19/LConn24
  Process_64/RConn10 -- Process_21/LConn17
  Process_64/RConn11 -- Process_26/LConn28
  Process_64/RConn12 -- Process_27/LConn27
  Process_64/RConn13 -- Process_29/LConn22
  Process_64/RConn14 -- Process_30/LConn24
  Process_64/RConn15 -- Process_33/LConn26
  Process_64/RConn16 -- Process_35/LConn22
  Process_64/RConn17 -- Process_40/LConn32
  Process_64/RConn18 -- Process_44/LConn27
  Process_64/RConn19 -- Process_46/LConn28
  Process_64/RConn20 -- Process_49/LConn25
  Process_64/RConn21 -- Process_51/LConn28
  Process_64/RConn22 -- Process_52/LConn24
  Process_64/RConn23 -- Process_54/LConn26
  Process_64/RConn24 -- Process_56/LConn30
  Process_64/RConn25 -- Process_63/LConn29
  Process_64/RConn26 -- Process_66/LConn24
  Process_64/RConn27 -- Process_67/LConn21
  Process_64/RConn28 -- Process_74/LConn21
  Process_64/RConn29 -- Process_75/LConn27
  Process_64/RConn30 -- Process_79/LConn28
  Process_64/RConn31 -- Process_84/LConn24
  Process_64/RConn32 -- Process_92/LConn24
  Process_64/RConn33 -- Process_93/LConn26
  Process_64/RConn34 -- Process_94/LConn25
  Process_64/RConn35 -- Process_96/LConn26
  Process_65/RConn1 -- Process_2/LConn20
  Process_65/RConn2 -- Process_4/LConn26
  Process_65/RConn3 -- Process_8/LConn25
  Process_65/RConn4 -- Process_9/LConn30
  Process_65/RConn5 -- Process_10/LConn24
  Process_65/RConn6 -- Process_19/LConn25
  Process_65/RConn7 -- Process_20/LConn20
  Process_65/RConn8 -- Process_21/LConn18
  Process_65/RConn9 -- Process_22/LConn23
  Process_65/RConn10 -- Process_26/LConn29
  Process_65/RConn11 -- Process_27/LConn28
  Process_65/RConn12 -- Process_28/LConn19
  Process_65/RConn13 -- Process_29/LConn23
  Process_65/RConn14 -- Process_32/LConn23
  Process_65/RConn15 -- Process_33/LConn27
  Process_65/RConn16 -- Process_36/LConn22
  Process_65/RConn17 -- Process_39/LConn20
  Process_65/RConn18 -- Process_45/LConn25
  Process_65/RConn19 -- Process_48/LConn26
  Process_65/RConn20 -- Process_49/LConn26
  Process_65/RConn21 -- Process_54/LConn27
  Process_65/RConn22 -- Process_56/LConn31
  Process_65/RConn23 -- Process_59/LConn31
  Process_65/RConn24 -- Process_60/LConn26
  Process_65/RConn25 -- Process_64/LConn25
  Process_65/RConn26 -- Process_65/LConn25
  Process_65/RConn27 -- Process_66/LConn25
  Process_65/RConn28 -- Process_69/LConn26
  Process_65/RConn29 -- Process_75/LConn28
  Process_65/RConn30 -- Process_77/LConn26
  Process_65/RConn31 -- Process_82/LConn24
  Process_65/RConn32 -- Process_88/LConn21
  Process_65/RConn33 -- Process_91/LConn26
  Process_65/RConn34 -- Process_93/LConn27
  Process_65/RConn35 -- Process_95/LConn18
  Process_65/RConn36 -- Process_98/LConn26
  Process_66/RConn1 -- Process_5/LConn19
  Process_66/RConn2 -- Process_6/LConn31
  Process_66/RConn3 -- Process_8/LConn26
  Process_66/RConn4 -- Process_9/LConn31
  Process_66/RConn5 -- Process_11/LConn33
  Process_66/RConn6 -- Process_16/LConn26
  Process_66/RConn7 -- Process_17/LConn28
  Process_66/RConn8 -- Process_19/LConn26
  Process_66/RConn9 -- Process_20/LConn21
  Process_66/RConn10 -- Process_23/LConn31
  Process_66/RConn11 -- Process_27/LConn29
  Process_66/RConn12 -- Process_28/LConn20
  Process_66/RConn13 -- Process_30/LConn25
  Process_66/RConn14 -- Process_31/LConn17
  Process_66/RConn15 -- Process_32/LConn24
  Process_66/RConn16 -- Process_34/LConn27
  Process_66/RConn17 -- Process_38/LConn27
  Process_66/RConn18 -- Process_39/LConn21
  Process_66/RConn19 -- Process_42/LConn25
  Process_66/RConn20 -- Process_47/LConn26
  Process_66/RConn21 -- Process_50/LConn29
  Process_66/RConn22 -- Process_58/LConn26
  Process_66/RConn23 -- Process_61/LConn28
  Process_66/RConn24 -- Process_63/LConn30
  Process_66/RConn25 -- Process_64/LConn26
  Process_66/RConn26 -- Process_66/LConn26
  Process_66/RConn27 -- Process_67/LConn22
  Process_66/RConn28 -- Process_68/LConn23
  Process_66/RConn29 -- Process_70/LConn21
  Process_66/RConn30 -- Process_73/LConn25
  Process_66/RConn31 -- Process_75/LConn29
  Process_66/RConn32 -- Process_76/LConn26
  Process_66/RConn33 -- Process_79/LConn29
  Process_66/RConn34 -- Process_82/LConn25
  Process_66/RConn35 -- Process_85/LConn27
  Process_66/RConn36 -- Process_86/LConn24
  Process_66/RConn37 -- Process_89/LConn27
  Process_66/RConn38 -- Process_90/LConn27
  Process_66/RConn39 -- Process_91/LConn27
  Process_66/RConn40 -- Process_92/LConn25
  Process_66/RConn41 -- Process_96/LConn27
  Process_67/RConn1 -- Process_9/LConn32
  Process_67/RConn2 -- Process_11/LConn34
  Process_67/RConn3 -- Process_12/LConn22
  Process_67/RConn4 -- Process_15/LConn21
  Process_67/RConn5 -- Process_20/LConn22
  Process_67/RConn6 -- Process_21/LConn19
  Process_67/RConn7 -- Process_24/LConn20
  Process_67/RConn8 -- Process_27/LConn30
  Process_67/RConn9 -- Process_29/LConn24
  Process_67/RConn10 -- Process_35/LConn23
  Process_67/RConn11 -- Process_36/LConn23
  Process_67/RConn12 -- Process_38/LConn28
  Process_67/RConn13 -- Process_39/LConn22
  Process_67/RConn14 -- Process_40/LConn33
  Process_67/RConn15 -- Process_41/LConn34
  Process_67/RConn16 -- Process_46/LConn29
  Process_67/RConn17 -- Process_47/LConn27
  Process_67/RConn18 -- Process_48/LConn27
  Process_67/RConn19 -- Process_49/LConn27
  Process_67/RConn20 -- Process_58/LConn27
  Process_67/RConn21 -- Process_59/LConn32
  Process_67/RConn22 -- Process_67/LConn23
  Process_67/RConn23 -- Process_71/LConn27
  Process_67/RConn24 -- Process_73/LConn26
  Process_67/RConn25 -- Process_82/LConn26
  Process_67/RConn26 -- Process_84/LConn25
  Process_67/RConn27 -- Process_85/LConn28
  Process_67/RConn28 -- Process_89/LConn28
  Process_67/RConn29 -- Process_92/LConn26
  Process_67/RConn30 -- Process_93/LConn28
  Process_67/RConn31 -- Process_94/LConn26
  Process_67/RConn32 -- Process_95/LConn19
  Process_67/RConn33 -- Process_97/LConn17
  Process_67/RConn34 -- Process_100/LConn23
  Process_68/RConn1 -- Process_2/LConn21
  Process_68/RConn2 -- Process_3/LConn22
  Process_68/RConn3 -- Process_4/LConn27
  Process_68/RConn4 -- Process_6/LConn32
  Process_68/RConn5 -- Process_7/LConn30
  Process_68/RConn6 -- Process_8/LConn27
  Process_68/RConn7 -- Process_9/LConn33
  Process_68/RConn8 -- Process_11/LConn35
  Process_68/RConn9 -- Process_12/LConn23
  Process_68/RConn10 -- Process_14/LConn27
  Process_68/RConn11 -- Process_15/LConn22
  Process_68/RConn12 -- Process_16/LConn27
  Process_68/RConn13 -- Process_17/LConn29
  Process_68/RConn14 -- Process_22/LConn24
  Process_68/RConn15 -- Process_24/LConn21
  Process_68/RConn16 -- Process_27/LConn31
  Process_68/RConn17 -- Process_30/LConn26
  Process_68/RConn18 -- Process_31/LConn18
  Process_68/RConn19 -- Process_32/LConn25
  Process_68/RConn20 -- Process_35/LConn24
  Process_68/RConn21 -- Process_37/LConn22
  Process_68/RConn22 -- Process_42/LConn26
  Process_68/RConn23 -- Process_43/LConn27
  Process_68/RConn24 -- Process_50/LConn30
  Process_68/RConn25 -- Process_56/LConn32
  Process_68/RConn26 -- Process_58/LConn28
  Process_68/RConn27 -- Process_62/LConn23
  Process_68/RConn28 -- Process_63/LConn31
  Process_68/RConn29 -- Process_68/LConn24
  Process_68/RConn30 -- Process_71/LConn28
  Process_68/RConn31 -- Process_72/LConn17
  Process_68/RConn32 -- Process_73/LConn27
  Process_68/RConn33 -- Process_78/LConn22
  Process_68/RConn34 -- Process_80/LConn18
  Process_68/RConn35 -- Process_81/LConn25
  Process_68/RConn36 -- Process_82/LConn27
  Process_68/RConn37 -- Process_83/LConn29
  Process_68/RConn38 -- Process_87/LConn26
  Process_68/RConn39 -- Process_90/LConn28
  Process_68/RConn40 -- Process_91/LConn28
  Process_68/RConn41 -- Process_99/LConn32
  Process_68/RConn42 -- Process_100/LConn24
  Process_69/RConn1 -- Process_1/LConn22
  Process_69/RConn2 -- Process_6/LConn33
  Process_69/RConn3 -- Process_10/LConn25
  Process_69/RConn4 -- Process_19/LConn27
  Process_69/RConn5 -- Process_20/LConn23
  Process_69/RConn6 -- Process_21/LConn20
  Process_69/RConn7 -- Process_22/LConn25
  Process_69/RConn8 -- Process_24/LConn22
  Process_69/RConn9 -- Process_25/LConn24
  Process_69/RConn10 -- Process_27/LConn32
  Process_69/RConn11 -- Process_30/LConn27
  Process_69/RConn12 -- Process_31/LConn19
  Process_69/RConn13 -- Process_33/LConn28
  Process_69/RConn14 -- Process_34/LConn28
  Process_69/RConn15 -- Process_36/LConn24
  Process_69/RConn16 -- Process_39/LConn23
  Process_69/RConn17 -- Process_40/LConn34
  Process_69/RConn18 -- Process_43/LConn28
  Process_69/RConn19 -- Process_48/LConn28
  Process_69/RConn20 -- Process_50/LConn31
  Process_69/RConn21 -- Process_56/LConn33
  Process_69/RConn22 -- Process_59/LConn33
  Process_69/RConn23 -- Process_62/LConn24
  Process_69/RConn24 -- Process_63/LConn32
  Process_69/RConn25 -- Process_65/LConn26
  Process_69/RConn26 -- Process_68/LConn25
  Process_69/RConn27 -- Process_69/LConn27
  Process_69/RConn28 -- Process_75/LConn30
  Process_69/RConn29 -- Process_76/LConn27
  Process_69/RConn30 -- Process_77/LConn27
  Process_69/RConn31 -- Process_78/LConn23
  Process_69/RConn32 -- Process_79/LConn30
  Process_69/RConn33 -- Process_80/LConn19
  Process_69/RConn34 -- Process_83/LConn30
  Process_69/RConn35 -- Process_89/LConn29
  Process_69/RConn36 -- Process_90/LConn29
  Process_69/RConn37 -- Process_91/LConn29
  Process_69/RConn38 -- Process_97/LConn18
  Process_69/RConn39 -- Process_98/LConn27
  Process_69/RConn40 -- Process_100/LConn25
  Process_70/RConn1 -- Process_2/LConn22
  Process_70/RConn2 -- Process_5/LConn20
  Process_70/RConn3 -- Process_7/LConn31
  Process_70/RConn4 -- Process_10/LConn26
  Process_70/RConn5 -- Process_12/LConn24
  Process_70/RConn6 -- Process_18/LConn28
  Process_70/RConn7 -- Process_19/LConn28
  Process_70/RConn8 -- Process_25/LConn25
  Process_70/RConn9 -- Process_26/LConn30
  Process_70/RConn10 -- Process_28/LConn21
  Process_70/RConn11 -- Process_29/LConn25
  Process_70/RConn12 -- Process_39/LConn24
  Process_70/RConn13 -- Process_45/LConn26
  Process_70/RConn14 -- Process_46/LConn30
  Process_70/RConn15 -- Process_48/LConn29
  Process_70/RConn16 -- Process_50/LConn32
  Process_70/RConn17 -- Process_54/LConn28
  Process_70/RConn18 -- Process_55/LConn34
  Process_70/RConn19 -- Process_61/LConn29
  Process_70/RConn20 -- Process_64/LConn27
  Process_70/RConn21 -- Process_66/LConn27
  Process_70/RConn22 -- Process_67/LConn24
  Process_70/RConn23 -- Process_68/LConn26
  Process_70/RConn24 -- Process_72/LConn18
  Process_70/RConn25 -- Process_73/LConn28
  Process_70/RConn26 -- Process_74/LConn22
  Process_70/RConn27 -- Process_76/LConn28
  Process_70/RConn28 -- Process_83/LConn31
  Process_70/RConn29 -- Process_84/LConn26
  Process_70/RConn30 -- Process_86/LConn25
  Process_70/RConn31 -- Process_88/LConn22
  Process_70/RConn32 -- Process_90/LConn30
  Process_70/RConn33 -- Process_91/LConn30
  Process_70/RConn34 -- Process_95/LConn20
  Process_70/RConn35 -- Process_96/LConn28
  Process_70/RConn36 -- Process_98/LConn28
  Process_71/RConn1 -- Process_3/LConn23
  Process_71/RConn2 -- Process_4/LConn28
  Process_71/RConn3 -- Process_5/LConn21
  Process_71/RConn4 -- Process_6/LConn34
  Process_71/RConn5 -- Process_10/LConn27
  Process_71/RConn6 -- Process_12/LConn25
  Process_71/RConn7 -- Process_13/LConn27
  Process_71/RConn8 -- Process_14/LConn28
  Process_71/RConn9 -- Process_15/LConn23
  Process_71/RConn10 -- Process_17/LConn30
  Process_71/RConn11 -- Process_19/LConn29
  Process_71/RConn12 -- Process_24/LConn23
  Process_71/RConn13 -- Process_26/LConn31
  Process_71/RConn14 -- Process_28/LConn22
  Process_71/RConn15 -- Process_33/LConn29
  Process_71/RConn16 -- Process_34/LConn29
  Process_71/RConn17 -- Process_39/LConn25
  Process_71/RConn18 -- Process_44/LConn28
  Process_71/RConn19 -- Process_45/LConn27
  Process_71/RConn20 -- Process_51/LConn29
  Process_71/RConn21 -- Process_52/LConn25
  Process_71/RConn22 -- Process_58/LConn29
  Process_71/RConn23 -- Process_60/LConn27
  Process_71/RConn24 -- Process_62/LConn25
  Process_71/RConn25 -- Process_64/LConn28
  Process_71/RConn26 -- Process_65/LConn27
  Process_71/RConn27 -- Process_66/LConn28
  Process_71/RConn28 -- Process_67/LConn25
  Process_71/RConn29 -- Process_68/LConn27
  Process_71/RConn30 -- Process_73/LConn29
  Process_71/RConn31 -- Process_75/LConn31
  Process_71/RConn32 -- Process_76/LConn29
  Process_71/RConn33 -- Process_77/LConn28
  Process_71/RConn34 -- Process_82/LConn28
  Process_71/RConn35 -- Process_83/LConn32
  Process_71/RConn36 -- Process_84/LConn27
  Process_71/RConn37 -- Process_85/LConn29
  Process_71/RConn38 -- Process_89/LConn30
  Process_71/RConn39 -- Process_91/LConn31
  Process_71/RConn40 -- Process_94/LConn27
  Process_71/RConn41 -- Process_98/LConn29
  Process_72/RConn1 -- Process_2/LConn23
  Process_72/RConn2 -- Process_5/LConn22
  Process_72/RConn3 -- Process_7/LConn32
  Process_72/RConn4 -- Process_12/LConn26
  Process_72/RConn5 -- Process_13/LConn28
  Process_72/RConn6 -- Process_16/LConn28
  Process_72/RConn7 -- Process_17/LConn31
  Process_72/RConn8 -- Process_18/LConn29
  Process_72/RConn9 -- Process_21/LConn21
  Process_72/RConn10 -- Process_31/LConn20
  Process_72/RConn11 -- Process_38/LConn29
  Process_72/RConn12 -- Process_39/LConn26
  Process_72/RConn13 -- Process_40/LConn35
  Process_72/RConn14 -- Process_43/LConn29
  Process_72/RConn15 -- Process_47/LConn28
  Process_72/RConn16 -- Process_50/LConn33
  Process_72/RConn17 -- Process_51/LConn30
  Process_72/RConn18 -- Process_52/LConn26
  Process_72/RConn19 -- Process_55/LConn35
  Process_72/RConn20 -- Process_57/LConn21
  Process_72/RConn21 -- Process_58/LConn30
  Process_72/RConn22 -- Process_61/LConn30
  Process_72/RConn23 -- Process_68/LConn28
  Process_72/RConn24 -- Process_70/LConn22
  Process_72/RConn25 -- Process_77/LConn29
  Process_72/RConn26 -- Process_82/LConn29
  Process_72/RConn27 -- Process_83/LConn33
  Process_72/RConn28 -- Process_84/LConn28
  Process_72/RConn29 -- Process_89/LConn31
  Process_72/RConn30 -- Process_90/LConn31
  Process_72/RConn31 -- Process_92/LConn27
  Process_72/RConn32 -- Process_94/LConn28
  Process_72/RConn33 -- Process_96/LConn29
  Process_72/RConn34 -- Process_99/LConn33
  Process_73/RConn1 -- Process_2/LConn24
  Process_73/RConn2 -- Process_3/LConn24
  Process_73/RConn3 -- Process_4/LConn29
  Process_73/RConn4 -- Process_6/LConn35
  Process_73/RConn5 -- Process_13/LConn29
  Process_73/RConn6 -- Process_14/LConn29
  Process_73/RConn7 -- Process_15/LConn24
  Process_73/RConn8 -- Process_16/LConn29
  Process_73/RConn9 -- Process_17/LConn32
  Process_73/RConn10 -- Process_19/LConn30
  Process_73/RConn11 -- Process_21/LConn22
  Process_73/RConn12 -- Process_22/LConn26
  Process_73/RConn13 -- Process_24/LConn24
  Process_73/RConn14 -- Process_26/LConn32
  Process_73/RConn15 -- Process_39/LConn27
  Process_73/RConn16 -- Process_41/LConn35
  Process_73/RConn17 -- Process_42/LConn27
  Process_73/RConn18 -- Process_44/LConn29
  Process_73/RConn19 -- Process_45/LConn28
  Process_73/RConn20 -- Process_49/LConn28
  Process_73/RConn21 -- Process_50/LConn34
  Process_73/RConn22 -- Process_51/LConn31
  Process_73/RConn23 -- Process_52/LConn27
  Process_73/RConn24 -- Process_54/LConn29
  Process_73/RConn25 -- Process_57/LConn22
  Process_73/RConn26 -- Process_58/LConn31
  Process_73/RConn27 -- Process_61/LConn31
  Process_73/RConn28 -- Process_67/LConn26
  Process_73/RConn29 -- Process_68/LConn29
  Process_73/RConn30 -- Process_69/LConn28
  Process_73/RConn31 -- Process_70/LConn23
  Process_73/RConn32 -- Process_71/LConn29
  Process_73/RConn33 -- Process_72/LConn19
  Process_73/RConn34 -- Process_74/LConn23
  Process_73/RConn35 -- Process_79/LConn31
  Process_73/RConn36 -- Process_80/LConn20
  Process_73/RConn37 -- Process_82/LConn30
  Process_73/RConn38 -- Process_89/LConn32
  Process_73/RConn39 -- Process_94/LConn29
  Process_73/RConn40 -- Process_95/LConn21
  Process_73/RConn41 -- Process_96/LConn30
  Process_73/RConn42 -- Process_97/LConn19
  Process_73/RConn43 -- Process_99/LConn34
  Process_74/RConn1 -- Process_4/LConn30
  Process_74/RConn2 -- Process_5/LConn23
  Process_74/RConn3 -- Process_6/LConn36
  Process_74/RConn4 -- Process_13/LConn30
  Process_74/RConn5 -- Process_15/LConn25
  Process_74/RConn6 -- Process_16/LConn30
  Process_74/RConn7 -- Process_21/LConn23
  Process_74/RConn8 -- Process_27/LConn33
  Process_74/RConn9 -- Process_30/LConn28
  Process_74/RConn10 -- Process_31/LConn21
  Process_74/RConn11 -- Process_34/LConn30
  Process_74/RConn12 -- Process_35/LConn25
  Process_74/RConn13 -- Process_37/LConn23
  Process_74/RConn14 -- Process_38/LConn30
  Process_74/RConn15 -- Process_44/LConn30
  Process_74/RConn16 -- Process_52/LConn28
  Process_74/RConn17 -- Process_54/LConn30
  Process_74/RConn18 -- Process_55/LConn36
  Process_74/RConn19 -- Process_58/LConn32
  Process_74/RConn20 -- Process_61/LConn32
  Process_74/RConn21 -- Process_67/LConn27
  Process_74/RConn22 -- Process_68/LConn30
  Process_74/RConn23 -- Process_69/LConn29
  Process_74/RConn24 -- Process_73/LConn30
  Process_74/RConn25 -- Process_81/LConn26
  Process_74/RConn26 -- Process_83/LConn34
  Process_74/RConn27 -- Process_86/LConn26
  Process_74/RConn28 -- Process_87/LConn27
  Process_74/RConn29 -- Process_88/LConn23
  Process_74/RConn30 -- Process_91/LConn32
  Process_74/RConn31 -- Process_94/LConn30
  Process_74/RConn32 -- Process_95/LConn22
  Process_74/RConn33 -- Process_98/LConn30
  Process_74/RConn34 -- Process_99/LConn35
  Process_75/RConn1 -- Process_2/LConn25
  Process_75/RConn2 -- Process_5/LConn24
  Process_75/RConn3 -- Process_10/LConn28
  Process_75/RConn4 -- Process_11/LConn36
  Process_75/RConn5 -- Process_12/LConn27
  Process_75/RConn6 -- Process_13/LConn31
  Process_75/RConn7 -- Process_15/LConn26
  Process_75/RConn8 -- Process_16/LConn31
  Process_75/RConn9 -- Process_17/LConn33
  Process_75/RConn10 -- Process_19/LConn31
  Process_75/RConn11 -- Process_20/LConn24
  Process_75/RConn12 -- Process_21/LConn24
  Process_75/RConn13 -- Process_23/LConn32
  Process_75/RConn14 -- Process_24/LConn25
  Process_75/RConn15 -- Process_25/LConn26
  Process_75/RConn16 -- Process_27/LConn34
  Process_75/RConn17 -- Process_28/LConn23
  Process_75/RConn18 -- Process_29/LConn26
  Process_75/RConn19 -- Process_30/LConn29
  Process_75/RConn20 -- Process_33/LConn30
  Process_75/RConn21 -- Process_35/LConn26
  Process_75/RConn22 -- Process_37/LConn24
  Process_75/RConn23 -- Process_40/LConn36
  Process_75/RConn24 -- Process_41/LConn36
  Process_75/RConn25 -- Process_44/LConn31
  Process_75/RConn26 -- Process_51/LConn32
  Process_75/RConn27 -- Process_53/LConn23
  Process_75/RConn28 -- Process_55/LConn37
  Process_75/RConn29 -- Process_56/LConn34
  Process_75/RConn30 -- Process_58/LConn33
  Process_75/RConn31 -- Process_59/LConn34
  Process_75/RConn32 -- Process_61/LConn33
  Process_75/RConn33 -- Process_62/LConn26
  Process_75/RConn34 -- Process_63/LConn33
  Process_75/RConn35 -- Process_65/LConn28
  Process_75/RConn36 -- Process_67/LConn28
  Process_75/RConn37 -- Process_71/LConn30
  Process_75/RConn38 -- Process_72/LConn20
  Process_75/RConn39 -- Process_74/LConn24
  Process_75/RConn40 -- Process_75/LConn32
  Process_75/RConn41 -- Process_79/LConn32
  Process_75/RConn42 -- Process_83/LConn35
  Process_75/RConn43 -- Process_84/LConn29
  Process_75/RConn44 -- Process_87/LConn28
  Process_75/RConn45 -- Process_88/LConn24
  Process_75/RConn46 -- Process_89/LConn33
  Process_75/RConn47 -- Process_90/LConn32
  Process_75/RConn48 -- Process_92/LConn28
  Process_75/RConn49 -- Process_93/LConn29
  Process_76/RConn1 -- Process_1/LConn23
  Process_76/RConn2 -- Process_2/LConn26
  Process_76/RConn3 -- Process_3/LConn25
  Process_76/RConn4 -- Process_5/LConn25
  Process_76/RConn5 -- Process_8/LConn28
  Process_76/RConn6 -- Process_9/LConn34
  Process_76/RConn7 -- Process_14/LConn30
  Process_76/RConn8 -- Process_15/LConn27
  Process_76/RConn9 -- Process_18/LConn30
  Process_76/RConn10 -- Process_20/LConn25
  Process_76/RConn11 -- Process_22/LConn27
  Process_76/RConn12 -- Process_24/LConn26
  Process_76/RConn13 -- Process_25/LConn27
  Process_76/RConn14 -- Process_29/LConn27
  Process_76/RConn15 -- Process_30/LConn30
  Process_76/RConn16 -- Process_31/LConn22
  Process_76/RConn17 -- Process_33/LConn31
  Process_76/RConn18 -- Process_37/LConn25
  Process_76/RConn19 -- Process_39/LConn28
  Process_76/RConn20 -- Process_41/LConn37
  Process_76/RConn21 -- Process_46/LConn31
  Process_76/RConn22 -- Process_50/LConn35
  Process_76/RConn23 -- Process_52/LConn29
  Process_76/RConn24 -- Process_53/LConn24
  Process_76/RConn25 -- Process_57/LConn23
  Process_76/RConn26 -- Process_60/LConn28
  Process_76/RConn27 -- Process_66/LConn29
  Process_76/RConn28 -- Process_76/LConn30
  Process_76/RConn29 -- Process_80/LConn21
  Process_76/RConn30 -- Process_83/LConn36
  Process_76/RConn31 -- Process_84/LConn30
  Process_76/RConn32 -- Process_85/LConn30
  Process_76/RConn33 -- Process_88/LConn25
  Process_76/RConn34 -- Process_89/LConn34
  Process_76/RConn35 -- Process_90/LConn33
  Process_76/RConn36 -- Process_92/LConn29
  Process_76/RConn37 -- Process_96/LConn31
  Process_77/RConn1 -- Process_1/LConn24
  Process_77/RConn2 -- Process_6/LConn37
  Process_77/RConn3 -- Process_7/LConn33
  Process_77/RConn4 -- Process_8/LConn29
  Process_77/RConn5 -- Process_10/LConn29
  Process_77/RConn6 -- Process_13/LConn32
  Process_77/RConn7 -- Process_15/LConn28
  Process_77/RConn8 -- Process_17/LConn34
  Process_77/RConn9 -- Process_25/LConn28
  Process_77/RConn10 -- Process_26/LConn33
  Process_77/RConn11 -- Process_29/LConn28
  Process_77/RConn12 -- Process_37/LConn26
  Process_77/RConn13 -- Process_39/LConn29
  Process_77/RConn14 -- Process_42/LConn28
  Process_77/RConn15 -- Process_45/LConn29
  Process_77/RConn16 -- Process_49/LConn29
  Process_77/RConn17 -- Process_51/LConn33
  Process_77/RConn18 -- Process_53/LConn25
  Process_77/RConn19 -- Process_55/LConn38
  Process_77/RConn20 -- Process_59/LConn35
  Process_77/RConn21 -- Process_63/LConn34
  Process_77/RConn22 -- Process_68/LConn31
  Process_77/RConn23 -- Process_71/LConn31
  Process_77/RConn24 -- Process_72/LConn21
  Process_77/RConn25 -- Process_77/LConn30
  Process_77/RConn26 -- Process_79/LConn33
  Process_77/RConn27 -- Process_80/LConn22
  Process_77/RConn28 -- Process_82/LConn31
  Process_77/RConn29 -- Process_83/LConn37
  Process_77/RConn30 -- Process_84/LConn31
  Process_77/RConn31 -- Process_85/LConn31
  Process_77/RConn32 -- Process_86/LConn27
  Process_77/RConn33 -- Process_89/LConn35
  Process_77/RConn34 -- Process_90/LConn34
  Process_77/RConn35 -- Process_98/LConn31
  Process_77/RConn36 -- Process_99/LConn36
  Process_77/RConn37 -- Process_100/LConn26
  Process_78/RConn1 -- Process_3/LConn26
  Process_78/RConn2 -- Process_5/LConn26
  Process_78/RConn3 -- Process_6/LConn38
  Process_78/RConn4 -- Process_7/LConn34
  Process_78/RConn5 -- Process_10/LConn30
  Process_78/RConn6 -- Process_13/LConn33
  Process_78/RConn7 -- Process_17/LConn35
  Process_78/RConn8 -- Process_18/LConn31
  Process_78/RConn9 -- Process_20/LConn26
  Process_78/RConn10 -- Process_22/LConn28
  Process_78/RConn11 -- Process_26/LConn34
  Process_78/RConn12 -- Process_35/LConn27
  Process_78/RConn13 -- Process_36/LConn25
  Process_78/RConn14 -- Process_37/LConn27
  Process_78/RConn15 -- Process_44/LConn32
  Process_78/RConn16 -- Process_46/LConn32
  Process_78/RConn17 -- Process_50/LConn36
  Process_78/RConn18 -- Process_56/LConn35
  Process_78/RConn19 -- Process_63/LConn35
  Process_78/RConn20 -- Process_65/LConn29
  Process_78/RConn21 -- Process_71/LConn32
  Process_78/RConn22 -- Process_72/LConn22
  Process_78/RConn23 -- Process_75/LConn33
  Process_78/RConn24 -- Process_78/LConn24
  Process_78/RConn25 -- Process_82/LConn32
  Process_78/RConn26 -- Process_84/LConn32
  Process_78/RConn27 -- Process_93/LConn30
  Process_78/RConn28 -- Process_94/LConn31
  Process_78/RConn29 -- Process_100/LConn27
  Process_79/RConn1 -- Process_4/LConn31
  Process_79/RConn2 -- Process_10/LConn31
  Process_79/RConn3 -- Process_12/LConn28
  Process_79/RConn4 -- Process_15/LConn29
  Process_79/RConn5 -- Process_18/LConn32
  Process_79/RConn6 -- Process_20/LConn27
  Process_79/RConn7 -- Process_21/LConn25
  Process_79/RConn8 -- Process_22/LConn29
  Process_79/RConn9 -- Process_27/LConn35
  Process_79/RConn10 -- Process_32/LConn26
  Process_79/RConn11 -- Process_35/LConn28
  Process_79/RConn12 -- Process_36/LConn26
  Process_79/RConn13 -- Process_41/LConn38
  Process_79/RConn14 -- Process_44/LConn33
  Process_79/RConn15 -- Process_46/LConn33
  Process_79/RConn16 -- Process_48/LConn30
  Process_79/RConn17 -- Process_53/LConn26
  Process_79/RConn18 -- Process_65/LConn30
  Process_79/RConn19 -- Process_66/LConn30
  Process_79/RConn20 -- Process_68/LConn32
  Process_79/RConn21 -- Process_69/LConn30
  Process_79/RConn22 -- Process_70/LConn24
  Process_79/RConn23 -- Process_71/LConn33
  Process_79/RConn24 -- Process_72/LConn23
  Process_79/RConn25 -- Process_73/LConn31
  Process_79/RConn26 -- Process_75/LConn34
  Process_79/RConn27 -- Process_76/LConn31
  Process_79/RConn28 -- Process_77/LConn31
  Process_79/RConn29 -- Process_82/LConn33
  Process_79/RConn30 -- Process_83/LConn38
  Process_79/RConn31 -- Process_84/LConn33
  Process_79/RConn32 -- Process_85/LConn32
  Process_79/RConn33 -- Process_89/LConn36
  Process_79/RConn34 -- Process_92/LConn30
  Process_79/RConn35 -- Process_93/LConn31
  Process_79/RConn36 -- Process_94/LConn32
  Process_79/RConn37 -- Process_97/LConn20
  Process_79/RConn38 -- Process_99/LConn37
  Process_80/RConn1 -- Process_4/LConn32
  Process_80/RConn2 -- Process_6/LConn39
  Process_80/RConn3 -- Process_7/LConn35
  Process_80/RConn4 -- Process_11/LConn37
  Process_80/RConn5 -- Process_13/LConn34
  Process_80/RConn6 -- Process_14/LConn31
  Process_80/RConn7 -- Process_15/LConn30
  Process_80/RConn8 -- Process_19/LConn32
  Process_80/RConn9 -- Process_20/LConn28
  Process_80/RConn10 -- Process_21/LConn26
  Process_80/RConn11 -- Process_22/LConn30
  Process_80/RConn12 -- Process_29/LConn29
  Process_80/RConn13 -- Process_31/LConn23
  Process_80/RConn14 -- Process_33/LConn32
  Process_80/RConn15 -- Process_36/LConn27
  Process_80/RConn16 -- Process_37/LConn28
  Process_80/RConn17 -- Process_38/LConn31
  Process_80/RConn18 -- Process_39/LConn30
  Process_80/RConn19 -- Process_41/LConn39
  Process_80/RConn20 -- Process_47/LConn29
  Process_80/RConn21 -- Process_50/LConn37
  Process_80/RConn22 -- Process_54/LConn31
  Process_80/RConn23 -- Process_58/LConn34
  Process_80/RConn24 -- Process_63/LConn36
  Process_80/RConn25 -- Process_64/LConn29
  Process_80/RConn26 -- Process_66/LConn31
  Process_80/RConn27 -- Process_68/LConn33
  Process_80/RConn28 -- Process_75/LConn35
  Process_80/RConn29 -- Process_76/LConn32
  Process_80/RConn30 -- Process_77/LConn32
  Process_80/RConn31 -- Process_80/LConn23
  Process_80/RConn32 -- Process_81/LConn27
  Process_80/RConn33 -- Process_84/LConn34
  Process_80/RConn34 -- Process_86/LConn28
  Process_80/RConn35 -- Process_87/LConn29
  Process_80/RConn36 -- Process_90/LConn35
  Process_80/RConn37 -- Process_91/LConn33
  Process_80/RConn38 -- Process_94/LConn33
  Process_80/RConn39 -- Process_95/LConn23
  Process_80/RConn40 -- Process_100/LConn28
  Process_81/RConn1 -- Process_12/LConn29
  Process_81/RConn2 -- Process_15/LConn31
  Process_81/RConn3 -- Process_16/LConn32
  Process_81/RConn4 -- Process_17/LConn36
  Process_81/RConn5 -- Process_18/LConn33
  Process_81/RConn6 -- Process_26/LConn35
  Process_81/RConn7 -- Process_29/LConn30
  Process_81/RConn8 -- Process_32/LConn27
  Process_81/RConn9 -- Process_33/LConn33
  Process_81/RConn10 -- Process_34/LConn31
  Process_81/RConn11 -- Process_40/LConn37
  Process_81/RConn12 -- Process_41/LConn40
  Process_81/RConn13 -- Process_42/LConn29
  Process_81/RConn14 -- Process_46/LConn34
  Process_81/RConn15 -- Process_48/LConn31
  Process_81/RConn16 -- Process_49/LConn30
  Process_81/RConn17 -- Process_50/LConn38
  Process_81/RConn18 -- Process_54/LConn32
  Process_81/RConn19 -- Process_68/LConn34
  Process_81/RConn20 -- Process_69/LConn31
  Process_81/RConn21 -- Process_71/LConn34
  Process_81/RConn22 -- Process_73/LConn32
  Process_81/RConn23 -- Process_74/LConn25
  Process_81/RConn24 -- Process_77/LConn33
  Process_81/RConn25 -- Process_81/LConn28
  Process_81/RConn26 -- Process_82/LConn34
  Process_81/RConn27 -- Process_84/LConn35
  Process_81/RConn28 -- Process_85/LConn33
  Process_81/RConn29 -- Process_89/LConn37
  Process_81/RConn30 -- Process_90/LConn36
  Process_81/RConn31 -- Process_91/LConn34
  Process_81/RConn32 -- Process_92/LConn31
  Process_81/RConn33 -- Process_94/LConn34
  Process_81/RConn34 -- Process_95/LConn24
  Process_81/RConn35 -- Process_96/LConn32
  Process_81/RConn36 -- Process_98/LConn32
  Process_81/RConn37 -- Process_100/LConn29
  Process_82/RConn1 -- Process_3/LConn27
  Process_82/RConn2 -- Process_13/LConn35
  Process_82/RConn3 -- Process_15/LConn32
  Process_82/RConn4 -- Process_16/LConn33
  Process_82/RConn5 -- Process_19/LConn33
  Process_82/RConn6 -- Process_25/LConn29
  Process_82/RConn7 -- Process_28/LConn24
  Process_82/RConn8 -- Process_29/LConn31
  Process_82/RConn9 -- Process_30/LConn31
  Process_82/RConn10 -- Process_33/LConn34
  Process_82/RConn11 -- Process_35/LConn29
  Process_82/RConn12 -- Process_37/LConn29
  Process_82/RConn13 -- Process_40/LConn38
  Process_82/RConn14 -- Process_43/LConn30
  Process_82/RConn15 -- Process_44/LConn34
  Process_82/RConn16 -- Process_51/LConn34
  Process_82/RConn17 -- Process_53/LConn27
  Process_82/RConn18 -- Process_54/LConn33
  Process_82/RConn19 -- Process_55/LConn39
  Process_82/RConn20 -- Process_56/LConn36
  Process_82/RConn21 -- Process_57/LConn24
  Process_82/RConn22 -- Process_58/LConn35
  Process_82/RConn23 -- Process_60/LConn29
  Process_82/RConn24 -- Process_63/LConn37
  Process_82/RConn25 -- Process_65/LConn31
  Process_82/RConn26 -- Process_67/LConn29
  Process_82/RConn27 -- Process_68/LConn35
  Process_82/RConn28 -- Process_70/LConn25
  Process_82/RConn29 -- Process_73/LConn33
  Process_82/RConn30 -- Process_74/LConn26
  Process_82/RConn31 -- Process_80/LConn24
  Process_82/RConn32 -- Process_81/LConn29
  Process_82/RConn33 -- Process_85/LConn34
  Process_82/RConn34 -- Process_86/LConn29
  Process_82/RConn35 -- Process_89/LConn38
  Process_82/RConn36 -- Process_90/LConn37
  Process_82/RConn37 -- Process_97/LConn21
  Process_82/RConn38 -- Process_98/LConn33
  Process_82/RConn39 -- Process_99/LConn38
  Process_83/RConn1 -- Process_4/LConn33
  Process_83/RConn2 -- Process_7/LConn36
  Process_83/RConn3 -- Process_9/LConn35
  Process_83/RConn4 -- Process_11/LConn38
  Process_83/RConn5 -- Process_15/LConn33
  Process_83/RConn6 -- Process_16/LConn34
  Process_83/RConn7 -- Process_20/LConn29
  Process_83/RConn8 -- Process_21/LConn27
  Process_83/RConn9 -- Process_22/LConn31
  Process_83/RConn10 -- Process_23/LConn33
  Process_83/RConn11 -- Process_28/LConn25
  Process_83/RConn12 -- Process_29/LConn32
  Process_83/RConn13 -- Process_33/LConn35
  Process_83/RConn14 -- Process_36/LConn28
  Process_83/RConn15 -- Process_37/LConn30
  Process_83/RConn16 -- Process_40/LConn39
  Process_83/RConn17 -- Process_41/LConn41
  Process_83/RConn18 -- Process_43/LConn31
  Process_83/RConn19 -- Process_44/LConn35
  Process_83/RConn20 -- Process_45/LConn30
  Process_83/RConn21 -- Process_46/LConn35
  Process_83/RConn22 -- Process_49/LConn31
  Process_83/RConn23 -- Process_51/LConn35
  Process_83/RConn24 -- Process_53/LConn28
  Process_83/RConn25 -- Process_55/LConn40
  Process_83/RConn26 -- Process_58/LConn36
  Process_83/RConn27 -- Process_59/LConn36
  Process_83/RConn28 -- Process_61/LConn34
  Process_83/RConn29 -- Process_66/LConn32
  Process_83/RConn30 -- Process_69/LConn32
  Process_83/RConn31 -- Process_70/LConn26
  Process_83/RConn32 -- Process_72/LConn24
  Process_83/RConn33 -- Process_73/LConn34
  Process_83/RConn34 -- Process_74/LConn27
  Process_83/RConn35 -- Process_75/LConn36
  Process_83/RConn36 -- Process_79/LConn34
  Process_83/RConn37 -- Process_82/LConn35
  Process_83/RConn38 -- Process_87/LConn30
  Process_83/RConn39 -- Process_89/LConn39
  Process_83/RConn40 -- Process_93/LConn32
  Process_83/RConn41 -- Process_96/LConn33
  Process_83/RConn42 -- Process_97/LConn22
  Process_83/RConn43 -- Process_98/LConn34
  Process_83/RConn44 -- Process_99/LConn39
  Process_84/RConn1 -- Process_3/LConn28
  Process_84/RConn2 -- Process_6/LConn40
  Process_84/RConn3 -- Process_9/LConn36
  Process_84/RConn4 -- Process_11/LConn39
  Process_84/RConn5 -- Process_12/LConn30
  Process_84/RConn6 -- Process_14/LConn32
  Process_84/RConn7 -- Process_15/LConn34
  Process_84/RConn8 -- Process_17/LConn37
  Process_84/RConn9 -- Process_18/LConn34
  Process_84/RConn10 -- Process_22/LConn32
  Process_84/RConn11 -- Process_24/LConn27
  Process_84/RConn12 -- Process_29/LConn33
  Process_84/RConn13 -- Process_32/LConn28
  Process_84/RConn14 -- Process_33/LConn36
  Process_84/RConn15 -- Process_34/LConn32
  Process_84/RConn16 -- Process_36/LConn29
  Process_84/RConn17 -- Process_37/LConn31
  Process_84/RConn18 -- Process_40/LConn40
  Process_84/RConn19 -- Process_41/LConn42
  Process_84/RConn20 -- Process_44/LConn36
  Process_84/RConn21 -- Process_45/LConn31
  Process_84/RConn22 -- Process_52/LConn30
  Process_84/RConn23 -- Process_54/LConn34
  Process_84/RConn24 -- Process_55/LConn41
  Process_84/RConn25 -- Process_60/LConn30
  Process_84/RConn26 -- Process_61/LConn35
  Process_84/RConn27 -- Process_62/LConn27
  Process_84/RConn28 -- Process_66/LConn33
  Process_84/RConn29 -- Process_70/LConn27
  Process_84/RConn30 -- Process_72/LConn25
  Process_84/RConn31 -- Process_75/LConn37
  Process_84/RConn32 -- Process_76/LConn33
  Process_84/RConn33 -- Process_81/LConn30
  Process_84/RConn34 -- Process_86/LConn30
  Process_84/RConn35 -- Process_89/LConn40
  Process_84/RConn36 -- Process_90/LConn38
  Process_84/RConn37 -- Process_92/LConn32
  Process_84/RConn38 -- Process_93/LConn33
  Process_84/RConn39 -- Process_96/LConn34
  Process_85/RConn1 -- Process_3/LConn29
  Process_85/RConn2 -- Process_5/LConn27
  Process_85/RConn3 -- Process_11/LConn40
  Process_85/RConn4 -- Process_12/LConn31
  Process_85/RConn5 -- Process_15/LConn35
  Process_85/RConn6 -- Process_16/LConn35
  Process_85/RConn7 -- Process_18/LConn35
  Process_85/RConn8 -- Process_20/LConn30
  Process_85/RConn9 -- Process_21/LConn28
  Process_85/RConn10 -- Process_24/LConn28
  Process_85/RConn11 -- Process_30/LConn32
  Process_85/RConn12 -- Process_41/LConn43
  Process_85/RConn13 -- Process_43/LConn32
  Process_85/RConn14 -- Process_44/LConn37
  Process_85/RConn15 -- Process_45/LConn32
  Process_85/RConn16 -- Process_47/LConn30
  Process_85/RConn17 -- Process_48/LConn32
  Process_85/RConn18 -- Process_52/LConn31
  Process_85/RConn19 -- Process_53/LConn29
  Process_85/RConn20 -- Process_55/LConn42
  Process_85/RConn21 -- Process_57/LConn25
  Process_85/RConn22 -- Process_58/LConn37
  Process_85/RConn23 -- Process_62/LConn28
  Process_85/RConn24 -- Process_66/LConn34
  Process_85/RConn25 -- Process_69/LConn33
  Process_85/RConn26 -- Process_70/LConn28
  Process_85/RConn27 -- Process_73/LConn35
  Process_85/RConn28 -- Process_74/LConn28
  Process_85/RConn29 -- Process_80/LConn25
  Process_85/RConn30 -- Process_86/LConn31
  Process_85/RConn31 -- Process_88/LConn26
  Process_85/RConn32 -- Process_89/LConn41
  Process_85/RConn33 -- Process_91/LConn35
  Process_85/RConn34 -- Process_92/LConn33
  Process_85/RConn35 -- Process_94/LConn35
  Process_85/RConn36 -- Process_98/LConn35
  Process_85/RConn37 -- Process_99/LConn40
  Process_86/RConn1 -- Process_2/LConn27
  Process_86/RConn2 -- Process_9/LConn37
  Process_86/RConn3 -- Process_10/LConn32
  Process_86/RConn4 -- Process_12/LConn32
  Process_86/RConn5 -- Process_13/LConn36
